simulink model "Auto_mode"  (R2017a)
settings: Solver=VariableStepAuto  StartTime=0.0  StopTime=30  FixedStep=Ts  RelTol=1e-3  EnableMultiTasking=on
model workspace (MAT data in the model file):
  AC_ATTITUDE_ACCEL_Y_CONTROLLER_MAX_RADSS = Simulink.Signal
  AC_ATTITUDE_ACCEL_Y_CONTROLLER_MAX_RADSS.DataType = 'double'
  AC_ATTITUDE_ACCEL_Y_CONTROLLER_MAX_RADSS.Dimensions = 1
  AC_ATTITUDE_ACCEL_Y_CONTROLLER_MAX_RADSS.DimensionsMode = 'auto'
  AC_ATTITUDE_ACCEL_Y_CONTROLLER_MAX_RADSS.Complexity = 'real'
  AC_ATTITUDE_ACCEL_Y_CONTROLLER_MAX_RADSS.SampleTime = -1
  AC_ATTITUDE_ACCEL_Y_CONTROLLER_MAX_RADSS.SamplingMode = 'Sample based'
  AC_ATTITUDE_ACCEL_Y_CONTROLLER_MAX_RADSS.InitialValue = '0.5'
  AC_ATTITUDE_CONTROL_MAX = Simulink.Signal
  AC_ATTITUDE_CONTROL_MAX.DataType = 'double'
  AC_ATTITUDE_CONTROL_MAX.Dimensions = 1
  AC_ATTITUDE_CONTROL_MAX.DimensionsMode = 'auto'
  AC_ATTITUDE_CONTROL_MAX.Complexity = 'real'
  AC_ATTITUDE_CONTROL_MAX.SampleTime = -1
  AC_ATTITUDE_CONTROL_MAX.SamplingMode = 'Sample based'
  AC_ATTITUDE_CONTROL_MAX.InitialValue = '0.5'
  AC_ATTITUDE_THRUST_ERROR_ANGLE = Simulink.Signal
  AC_ATTITUDE_THRUST_ERROR_ANGLE.DataType = 'double'
  AC_ATTITUDE_THRUST_ERROR_ANGLE.Dimensions = 1
  AC_ATTITUDE_THRUST_ERROR_ANGLE.DimensionsMode = 'auto'
  AC_ATTITUDE_THRUST_ERROR_ANGLE.Complexity = 'real'
  AC_ATTITUDE_THRUST_ERROR_ANGLE.SampleTime = -1
  AC_ATTITUDE_THRUST_ERROR_ANGLE.SamplingMode = 'Sample based'
  AC_ATTITUDE_THRUST_ERROR_ANGLE.InitialValue = '1000'
  ROLL_PITCH_INPUT_MAX = Simulink.Signal
  ROLL_PITCH_INPUT_MAX.DataType = 'double'
  ROLL_PITCH_INPUT_MAX.Dimensions = 1
  ROLL_PITCH_INPUT_MAX.DimensionsMode = 'auto'
  ROLL_PITCH_INPUT_MAX.Complexity = 'real'
  ROLL_PITCH_INPUT_MAX.SampleTime = -1
  ROLL_PITCH_INPUT_MAX.SamplingMode = 'Sample based'
  ROLL_PITCH_INPUT_MAX.InitialValue = '3000'
  Sig = Simulink.Signal
  Sig.DataType = 'auto'
  Sig.Dimensions = -1
  Sig.DimensionsMode = 'auto'
  Sig.Complexity = 'auto'
  Sig.SampleTime = -1
  Sig.SamplingMode = 'auto'
  Sig1 = Simulink.Signal
  Sig1.DataType = 'auto'
  Sig1.Dimensions = -1
  Sig1.DimensionsMode = 'auto'
  Sig1.Complexity = 'auto'
  Sig1.SampleTime = -1
  Sig1.SamplingMode = 'auto'
  acro_yaw_p = Simulink.Signal
  acro_yaw_p.DataType = 'double'
  acro_yaw_p.Dimensions = 1
  acro_yaw_p.DimensionsMode = 'auto'
  acro_yaw_p.Complexity = 'real'
  acro_yaw_p.SampleTime = -1
  acro_yaw_p.SamplingMode = 'Sample based'
  acro_yaw_p.InitialValue = '45'
  angle_max = Simulink.Signal
  angle_max.DataType = 'double'
  angle_max.Dimensions = 1
  angle_max.DimensionsMode = 'auto'
  angle_max.Complexity = 'real'
  angle_max.SampleTime = -1
  angle_max.SamplingMode = 'Sample based'
  angle_max.InitialValue = '3000'
  attitude_target_ang_vel = Simulink.Signal
  attitude_target_ang_vel.DataType = 'double'
  attitude_target_ang_vel.Dimensions = 3
  attitude_target_ang_vel.DimensionsMode = 'auto'
  attitude_target_ang_vel.Complexity = 'real'
  attitude_target_ang_vel.SampleTime = -1
  attitude_target_ang_vel.SamplingMode = 'Sample based'
  attitude_target_ang_vel.InitialValue = '[0 0 0]'
  attitude_target_euler_angle_x = Simulink.Signal
  attitude_target_euler_angle_x.DataType = 'double'
  attitude_target_euler_angle_x.Dimensions = 1
  attitude_target_euler_angle_x.DimensionsMode = 'auto'
  attitude_target_euler_angle_x.Complexity = 'real'
  attitude_target_euler_angle_x.SampleTime = -1
  attitude_target_euler_angle_x.SamplingMode = 'Sample based'
  attitude_target_euler_angle_x.InitialValue = '0'
  attitude_target_euler_angle_y = Simulink.Signal
  attitude_target_euler_angle_y.DataType = 'double'
  attitude_target_euler_angle_y.Dimensions = 1
  attitude_target_euler_angle_y.DimensionsMode = 'auto'
  attitude_target_euler_angle_y.Complexity = 'real'
  attitude_target_euler_angle_y.SampleTime = -1
  attitude_target_euler_angle_y.SamplingMode = 'Sample based'
  attitude_target_euler_angle_y.InitialValue = '0'
  attitude_target_euler_angle_z = Simulink.Signal
  attitude_target_euler_angle_z.DataType = 'double'
  attitude_target_euler_angle_z.Dimensions = 1
  attitude_target_euler_angle_z.DimensionsMode = 'auto'
  attitude_target_euler_angle_z.Complexity = 'real'
  attitude_target_euler_angle_z.SampleTime = -1
  attitude_target_euler_angle_z.SamplingMode = 'Sample based'
  attitude_target_euler_angle_z.InitialValue = '0'
  attitude_target_euler_rate = Simulink.Signal
  attitude_target_euler_rate.DataType = 'double'
  attitude_target_euler_rate.Dimensions = 3
  attitude_target_euler_rate.DimensionsMode = 'auto'
  attitude_target_euler_rate.Complexity = 'real'
  attitude_target_euler_rate.SampleTime = -1
  attitude_target_euler_rate.SamplingMode = 'Sample based'
  attitude_target_euler_rate.InitialValue = '[0 0 0]'
  attitude_target_quat = Simulink.Signal
  attitude_target_quat.DataType = 'double'
  attitude_target_quat.Dimensions = 4
  attitude_target_quat.DimensionsMode = 'auto'
  attitude_target_quat.Complexity = 'real'
  attitude_target_quat.SampleTime = -1
  attitude_target_quat.SamplingMode = 'Sample based'
  attitude_target_quat.InitialValue = '[1 0 0 0]'
  attitude_vehicle_quat = Simulink.Signal
  attitude_vehicle_quat.DataType = 'double'
  attitude_vehicle_quat.Dimensions = 4
  attitude_vehicle_quat.DimensionsMode = 'auto'
  attitude_vehicle_quat.Complexity = 'real'
  attitude_vehicle_quat.SampleTime = -1
  attitude_vehicle_quat.SamplingMode = 'Sample based'
  attitude_vehicle_quat.InitialValue = '[1 0 0 0]'
  dt = Simulink.Signal
  dt.DataType = 'double'
  dt.Dimensions = 1
  dt.DimensionsMode = 'auto'
  dt.Complexity = 'real'
  dt.SampleTime = -1
  dt.SamplingMode = 'Sample based'
  dt.InitialValue = '0.01'
  false = 0
  limit_roll_pitch = Simulink.Signal
  limit_roll_pitch.DataType = 'double'
  limit_roll_pitch.Dimensions = 1
  limit_roll_pitch.DimensionsMode = 'auto'
  limit_roll_pitch.Complexity = 'real'
  limit_roll_pitch.SampleTime = -1
  limit_roll_pitch.SamplingMode = 'Sample based'
  limit_roll_pitch.InitialValue = '0.0'
  limit_throttle_upper = Simulink.Signal
  limit_throttle_upper.DataType = 'logical'
  limit_throttle_upper.Dimensions = 1
  limit_throttle_upper.DimensionsMode = 'auto'
  limit_throttle_upper.Complexity = 'real'
  limit_throttle_upper.SampleTime = -1
  limit_throttle_upper.SamplingMode = 'Sample based'
  limit_throttle_upper.InitialValue = '0'
  limit_yaw = Simulink.Signal
  limit_yaw.DataType = 'double'
  limit_yaw.Dimensions = 1
  limit_yaw.DimensionsMode = 'auto'
  limit_yaw.Complexity = 'real'
  limit_yaw.SampleTime = -1
  limit_yaw.SamplingMode = 'Sample based'
  limit_yaw.InitialValue = '0'
  loop_rate = Simulink.Signal
  loop_rate.DataType = 'double'
  loop_rate.Dimensions = 1
  loop_rate.DimensionsMode = 'auto'
  loop_rate.Complexity = 'real'
  loop_rate.SampleTime = -1
  loop_rate.SamplingMode = 'Sample based'
  loop_rate.InitialValue = '100'
  pitch_attitude_kP = Simulink.Signal
  pitch_attitude_kP.DataType = 'double'
  pitch_attitude_kP.Dimensions = 1
  pitch_attitude_kP.DimensionsMode = 'auto'
  pitch_attitude_kP.Complexity = 'real'
  pitch_attitude_kP.SampleTime = -1
  pitch_attitude_kP.SamplingMode = 'Sample based'
  pitch_attitude_kP.InitialValue = '20'
  pitch_factor = Simulink.Signal
  pitch_factor.DataType = 'double'
  pitch_factor.Dimensions = 4
  pitch_factor.DimensionsMode = 'auto'
  pitch_factor.Complexity = 'real'
  pitch_factor.SampleTime = -1
  pitch_factor.SamplingMode = 'Sample based'
  pitch_factor.InitialValue = '[cos(deg2rad(15)) -cos(deg2rad(15)) cos(deg2rad(15)) -cos(deg2rad(15))]'
  pitch_rate_derivative = Simulink.Signal
  pitch_rate_derivative.DataType = 'double'
  pitch_rate_derivative.Dimensions = 1
  pitch_rate_derivative.DimensionsMode = 'auto'
  pitch_rate_derivative.Complexity = 'real'
  pitch_rate_derivative.SampleTime = -1
  pitch_rate_derivative.SamplingMode = 'Sample based'
  pitch_rate_derivative.InitialValue = '0'
  pitch_rate_error_rads = Simulink.Signal
  pitch_rate_error_rads.DataType = 'double'
  pitch_rate_error_rads.Dimensions = 1
  pitch_rate_error_rads.DimensionsMode = 'auto'
  pitch_rate_error_rads.Complexity = 'real'
  pitch_rate_error_rads.SampleTime = -1
  pitch_rate_error_rads.SamplingMode = 'Sample based'
  pitch_rate_error_rads.InitialValue = '0'
  pitch_rate_filt_hz = Simulink.Signal
  pitch_rate_filt_hz.DataType = 'double'
  pitch_rate_filt_hz.Dimensions = 1
  pitch_rate_filt_hz.DimensionsMode = 'auto'
  pitch_rate_filt_hz.Complexity = 'real'
  pitch_rate_filt_hz.SampleTime = -1
  pitch_rate_filt_hz.SamplingMode = 'Sample based'
  pitch_rate_filt_hz.InitialValue = '1/(2*pi)'
  pitch_rate_imax = Simulink.Signal
  pitch_rate_imax.DataType = 'double'
  pitch_rate_imax.Dimensions = 1
  pitch_rate_imax.DimensionsMode = 'auto'
  pitch_rate_imax.Complexity = 'real'
  pitch_rate_imax.SampleTime = -1
  pitch_rate_imax.SamplingMode = 'Sample based'
  pitch_rate_imax.InitialValue = '200'
  pitch_rate_integrator = Simulink.Signal
  pitch_rate_integrator.DataType = 'double'
  pitch_rate_integrator.Dimensions = 1
  pitch_rate_integrator.DimensionsMode = 'auto'
  pitch_rate_integrator.Complexity = 'real'
  pitch_rate_integrator.SampleTime = -1
  pitch_rate_integrator.SamplingMode = 'Sample based'
  pitch_rate_integrator.InitialValue = '0'
  pitch_rate_kD = Simulink.Signal
  pitch_rate_kD.DataType = 'double'
  pitch_rate_kD.Dimensions = 1
  pitch_rate_kD.DimensionsMode = 'auto'
  pitch_rate_kD.Complexity = 'real'
  pitch_rate_kD.SampleTime = -1
  pitch_rate_kD.SamplingMode = 'Sample based'
  pitch_rate_kD.InitialValue = '0.004'
  pitch_rate_kI = Simulink.Signal
  pitch_rate_kI.DataType = 'double'
  pitch_rate_kI.Dimensions = 1
  pitch_rate_kI.DimensionsMode = 'auto'
  pitch_rate_kI.Complexity = 'real'
  pitch_rate_kI.SampleTime = -1
  pitch_rate_kI.SamplingMode = 'Sample based'
  pitch_rate_kI.InitialValue = '0.1'
  pitch_rate_kP = Simulink.Signal
  pitch_rate_kP.DataType = 'double'
  pitch_rate_kP.Dimensions = 1
  pitch_rate_kP.DimensionsMode = 'auto'
  pitch_rate_kP.Complexity = 'real'
  pitch_rate_kP.SampleTime = -1
  pitch_rate_kP.SamplingMode = 'Sample based'
  pitch_rate_kP.InitialValue = '0.5'
  pitch_rate_last_input = Simulink.Signal
  pitch_rate_last_input.DataType = 'double'
  pitch_rate_last_input.Dimensions = 1
  pitch_rate_last_input.DimensionsMode = 'auto'
  pitch_rate_last_input.Complexity = 'real'
  pitch_rate_last_input.SampleTime = -1
  pitch_rate_last_input.SamplingMode = 'Sample based'
  pitch_rate_last_input.InitialValue = '0'
  pitch_rate_proportional = Simulink.Signal
  pitch_rate_proportional.DataType = 'double'
  pitch_rate_proportional.Dimensions = 1
  pitch_rate_proportional.DimensionsMode = 'auto'
  pitch_rate_proportional.Complexity = 'real'
  pitch_rate_proportional.SampleTime = -1
  pitch_rate_proportional.SamplingMode = 'Sample based'
  pitch_rate_proportional.InitialValue = '0'
  pwm_max = Simulink.Signal
  pwm_max.DataType = 'double'
  pwm_max.Dimensions = 1
  pwm_max.DimensionsMode = 'auto'
  pwm_max.Complexity = 'real'
  pwm_max.SampleTime = -1
  pwm_max.SamplingMode = 'Sample based'
  pwm_max.InitialValue = '2000'
  pwm_min = Simulink.Signal
  pwm_min.DataType = 'double'
  pwm_min.Dimensions = 1
  pwm_min.DimensionsMode = 'auto'
  pwm_min.Complexity = 'real'
  pwm_min.SampleTime = -1
  pwm_min.SamplingMode = 'Sample based'
  pwm_min.InitialValue = '1039'
  rate_bf_ff_enabled = Simulink.Signal
  rate_bf_ff_enabled.DataType = 'double'
  rate_bf_ff_enabled.Dimensions = 1
  rate_bf_ff_enabled.DimensionsMode = 'auto'
  rate_bf_ff_enabled.Complexity = 'real'
  rate_bf_ff_enabled.SampleTime = -1
  rate_bf_ff_enabled.SamplingMode = 'Sample based'
  rate_bf_ff_enabled.InitialValue = '0'
  rate_target_ang_vel = Simulink.Signal
  rate_target_ang_vel.DataType = 'double'
  rate_target_ang_vel.Dimensions = 3
  rate_target_ang_vel.DimensionsMode = 'auto'
  rate_target_ang_vel.Complexity = 'real'
  rate_target_ang_vel.SampleTime = -1
  rate_target_ang_vel.SamplingMode = 'Sample based'
  rate_target_ang_vel.InitialValue = '[0 0 0]'
  roll_attitude_kP = Simulink.Signal
  roll_attitude_kP.DataType = 'double'
  roll_attitude_kP.Dimensions = 1
  roll_attitude_kP.DimensionsMode = 'auto'
  roll_attitude_kP.Complexity = 'real'
  roll_attitude_kP.SampleTime = -1
  roll_attitude_kP.SamplingMode = 'Sample based'
  roll_attitude_kP.InitialValue = '20'
  roll_factor = Simulink.Signal
  roll_factor.DataType = 'double'
  roll_factor.Dimensions = 4
  roll_factor.DimensionsMode = 'auto'
  roll_factor.Complexity = 'real'
  roll_factor.SampleTime = -1
  roll_factor.SamplingMode = 'Sample based'
  roll_factor.InitialValue = '[-sin(deg2rad(15)) sin(deg2rad(15)) sin(deg2rad(15)) -sin(deg2rad(15))]'
  roll_rate_derivative = Simulink.Signal
  roll_rate_derivative.DataType = 'double'
  roll_rate_derivative.Dimensions = 1
  roll_rate_derivative.DimensionsMode = 'auto'
  roll_rate_derivative.Complexity = 'real'
  roll_rate_derivative.SampleTime = -1
  roll_rate_derivative.SamplingMode = 'Sample based'
  roll_rate_derivative.InitialValue = '0'
  roll_rate_error_rads = Simulink.Signal
  roll_rate_error_rads.DataType = 'double'
  roll_rate_error_rads.Dimensions = 1
  roll_rate_error_rads.DimensionsMode = 'auto'
  roll_rate_error_rads.Complexity = 'real'
  roll_rate_error_rads.SampleTime = -1
  roll_rate_error_rads.SamplingMode = 'Sample based'
  roll_rate_error_rads.InitialValue = '0'
  roll_rate_filt_hz = Simulink.Signal
  roll_rate_filt_hz.DataType = 'double'
  roll_rate_filt_hz.Dimensions = 1
  roll_rate_filt_hz.DimensionsMode = 'auto'
  roll_rate_filt_hz.Complexity = 'real'
  roll_rate_filt_hz.SampleTime = -1
  roll_rate_filt_hz.SamplingMode = 'Sample based'
  roll_rate_filt_hz.InitialValue = '1/(2*pi)'
  roll_rate_imax = Simulink.Signal
  roll_rate_imax.DataType = 'double'
  roll_rate_imax.Dimensions = 1
  roll_rate_imax.DimensionsMode = 'auto'
  roll_rate_imax.Complexity = 'real'
  roll_rate_imax.SampleTime = -1
  roll_rate_imax.SamplingMode = 'Sample based'
  roll_rate_imax.InitialValue = '200'
  roll_rate_integrator = Simulink.Signal
  roll_rate_integrator.DataType = 'double'
  roll_rate_integrator.Dimensions = 1
  roll_rate_integrator.DimensionsMode = 'auto'
  roll_rate_integrator.Complexity = 'real'
  roll_rate_integrator.SampleTime = -1
  roll_rate_integrator.SamplingMode = 'Sample based'
  roll_rate_integrator.InitialValue = '0'
  roll_rate_kD = Simulink.Signal
  roll_rate_kD.DataType = 'double'
  roll_rate_kD.Dimensions = 1
  roll_rate_kD.DimensionsMode = 'auto'
  roll_rate_kD.Complexity = 'real'
  roll_rate_kD.SampleTime = -1
  roll_rate_kD.SamplingMode = 'Sample based'
  roll_rate_kD.InitialValue = '0.004'
  roll_rate_kI = Simulink.Signal
  roll_rate_kI.DataType = 'double'
  roll_rate_kI.Dimensions = 1
  roll_rate_kI.DimensionsMode = 'auto'
  roll_rate_kI.Complexity = 'real'
  roll_rate_kI.SampleTime = -1
  roll_rate_kI.SamplingMode = 'Sample based'
  roll_rate_kI.InitialValue = '0.1'
  roll_rate_kP = Simulink.Signal
  roll_rate_kP.DataType = 'double'
  roll_rate_kP.Dimensions = 1
  roll_rate_kP.DimensionsMode = 'auto'
  roll_rate_kP.Complexity = 'real'
  roll_rate_kP.SampleTime = -1
  roll_rate_kP.SamplingMode = 'Sample based'
  roll_rate_kP.InitialValue = '1'
  roll_rate_last_input = Simulink.Signal
  roll_rate_last_input.DataType = 'double'
  roll_rate_last_input.Dimensions = 1
  roll_rate_last_input.DimensionsMode = 'auto'
  roll_rate_last_input.Complexity = 'real'
  roll_rate_last_input.SampleTime = -1
  roll_rate_last_input.SamplingMode = 'Sample based'
  roll_rate_last_input.InitialValue = '0'
  roll_rate_proportional = Simulink.Signal
  roll_rate_proportional.DataType = 'double'
  roll_rate_proportional.Dimensions = 1
  roll_rate_proportional.DimensionsMode = 'auto'
  roll_rate_proportional.Complexity = 'real'
  roll_rate_proportional.SampleTime = -1
  roll_rate_proportional.SamplingMode = 'Sample based'
  roll_rate_proportional.InitialValue = '0'
  spin_max = Simulink.Signal
  spin_max.DataType = 'double'
  spin_max.Dimensions = 1
  spin_max.DimensionsMode = 'auto'
  spin_max.Complexity = 'real'
  spin_max.SampleTime = -1
  spin_max.SamplingMode = 'Sample based'
  spin_max.InitialValue = '0.95'
  spin_min = Simulink.Signal
  spin_min.DataType = 'double'
  spin_min.Dimensions = 1
  spin_min.DimensionsMode = 'auto'
  spin_min.Complexity = 'real'
  spin_min.SampleTime = -1
  spin_min.SamplingMode = 'Sample based'
  spin_min.InitialValue = '0.15'
  throttle_avg_max = Simulink.Signal
  throttle_avg_max.DataType = 'double'
  throttle_avg_max.Dimensions = 1
  throttle_avg_max.DimensionsMode = 'auto'
  throttle_avg_max.Complexity = 'real'
  throttle_avg_max.SampleTime = -1
  throttle_avg_max.SamplingMode = 'Sample based'
  throttle_avg_max.InitialValue = '0'
  throttle_filter_cutoff_freq = Simulink.Signal
  throttle_filter_cutoff_freq.DataType = 'double'
  throttle_filter_cutoff_freq.Dimensions = 1
  throttle_filter_cutoff_freq.DimensionsMode = 'auto'
  throttle_filter_cutoff_freq.Complexity = 'real'
  throttle_filter_cutoff_freq.SampleTime = -1
  throttle_filter_cutoff_freq.SamplingMode = 'Sample based'
  throttle_filter_cutoff_freq.InitialValue = '0.5'
  throttle_filter_output = Simulink.Signal
  throttle_filter_output.DataType = 'double'
  throttle_filter_output.Dimensions = 1
  throttle_filter_output.DimensionsMode = 'auto'
  throttle_filter_output.Complexity = 'real'
  throttle_filter_output.SampleTime = -1
  throttle_filter_output.SamplingMode = 'Sample based'
  throttle_filter_output.InitialValue = '0'
  throttle_in = Simulink.Signal
  throttle_in.DataType = 'double'
  throttle_in.Dimensions = 1
  throttle_in.DimensionsMode = 'auto'
  throttle_in.Complexity = 'real'
  throttle_in.SampleTime = -1
  throttle_in.SamplingMode = 'Sample based'
  throttle_in.InitialValue = '0'
  throttle_rpy_mix = Simulink.Signal
  throttle_rpy_mix.DataType = 'double'
  throttle_rpy_mix.Dimensions = 1
  throttle_rpy_mix.DimensionsMode = 'auto'
  throttle_rpy_mix.Complexity = 'real'
  throttle_rpy_mix.SampleTime = -1
  throttle_rpy_mix.SamplingMode = 'Sample based'
  throttle_rpy_mix.InitialValue = '0'
  throttle_rpy_mix_desired = Simulink.Signal
  throttle_rpy_mix_desired.DataType = 'double'
  throttle_rpy_mix_desired.Dimensions = 1
  throttle_rpy_mix_desired.DimensionsMode = 'auto'
  throttle_rpy_mix_desired.Complexity = 'real'
  throttle_rpy_mix_desired.SampleTime = -1
  throttle_rpy_mix_desired.SamplingMode = 'Sample based'
  throttle_rpy_mix_desired.InitialValue = '0'
  throttle_thrust = Simulink.Signal
  throttle_thrust.DataType = 'double'
  throttle_thrust.Dimensions = 1
  throttle_thrust.DimensionsMode = 'auto'
  throttle_thrust.Complexity = 'real'
  throttle_thrust.SampleTime = -1
  throttle_thrust.SamplingMode = 'Sample based'
  throttle_thrust.InitialValue = '0'
  throttle_thrust_best_rpy = Simulink.Signal
  throttle_thrust_best_rpy.DataType = 'double'
  throttle_thrust_best_rpy.Dimensions = 1
  throttle_thrust_best_rpy.DimensionsMode = 'auto'
  throttle_thrust_best_rpy.Complexity = 'real'
  throttle_thrust_best_rpy.SampleTime = -1
  throttle_thrust_best_rpy.SamplingMode = 'Sample based'
  throttle_thrust_best_rpy.InitialValue = '0'
  throttle_thrust_max = Simulink.Signal
  throttle_thrust_max.DataType = 'double'
  throttle_thrust_max.Dimensions = 1
  throttle_thrust_max.DimensionsMode = 'auto'
  throttle_thrust_max.Complexity = 'real'
  throttle_thrust_max.SampleTime = -1
  throttle_thrust_max.SamplingMode = 'Sample based'
  throttle_thrust_max.InitialValue = '1'
  thrust_error_angle = Simulink.Signal
  thrust_error_angle.DataType = 'double'
  thrust_error_angle.Dimensions = 1
  thrust_error_angle.DimensionsMode = 'auto'
  thrust_error_angle.Complexity = 'real'
  thrust_error_angle.SampleTime = -1
  thrust_error_angle.SamplingMode = 'Sample based'
  thrust_error_angle.InitialValue = '0'
  thrust_rpyt_out = Simulink.Signal
  thrust_rpyt_out.DataType = 'double'
  thrust_rpyt_out.Dimensions = 4
  thrust_rpyt_out.DimensionsMode = 'auto'
  thrust_rpyt_out.Complexity = 'real'
  thrust_rpyt_out.SampleTime = -1
  thrust_rpyt_out.SamplingMode = 'Sample based'
  thrust_rpyt_out.InitialValue = '[0 0 0 0]'
  true = 1
  use_ff_and_input_shaping = Simulink.Signal
  use_ff_and_input_shaping.DataType = 'double'
  use_ff_and_input_shaping.Dimensions = 1
  use_ff_and_input_shaping.DimensionsMode = 'auto'
  use_ff_and_input_shaping.Complexity = 'real'
  use_ff_and_input_shaping.SampleTime = -1
  use_ff_and_input_shaping.SamplingMode = 'Sample based'
  use_ff_and_input_shaping.InitialValue = '0'
  variableType = 'S'
  yaw_allowed = Simulink.Signal
  yaw_allowed.DataType = 'double'
  yaw_allowed.Dimensions = 1
  yaw_allowed.DimensionsMode = 'auto'
  yaw_allowed.Complexity = 'real'
  yaw_allowed.SampleTime = -1
  yaw_allowed.SamplingMode = 'Sample based'
  yaw_allowed.InitialValue = '1'
  yaw_attitude_kP = Simulink.Signal
  yaw_attitude_kP.DataType = 'double'
  yaw_attitude_kP.Dimensions = 1
  yaw_attitude_kP.DimensionsMode = 'auto'
  yaw_attitude_kP.Complexity = 'real'
  yaw_attitude_kP.SampleTime = -1
  yaw_attitude_kP.SamplingMode = 'Sample based'
  yaw_attitude_kP.InitialValue = '4.5'
  yaw_factor = Simulink.Signal
  yaw_factor.DataType = 'double'
  yaw_factor.Dimensions = 4
  yaw_factor.DimensionsMode = 'auto'
  yaw_factor.Complexity = 'real'
  yaw_factor.SampleTime = -1
  yaw_factor.SamplingMode = 'Sample based'
  yaw_factor.InitialValue = '[0.1 0.1 -0.1 -0.1]'
  yaw_headroom = Simulink.Signal
  yaw_headroom.DataType = 'double'
  yaw_headroom.Dimensions = 1
  yaw_headroom.DimensionsMode = 'auto'
  yaw_headroom.Complexity = 'real'
  yaw_headroom.SampleTime = -1
  yaw_headroom.SamplingMode = 'Sample based'
  yaw_headroom.InitialValue = '200'
  yaw_rate_derivative = Simulink.Signal
  yaw_rate_derivative.DataType = 'double'
  yaw_rate_derivative.Dimensions = 1
  yaw_rate_derivative.DimensionsMode = 'auto'
  yaw_rate_derivative.Complexity = 'real'
  yaw_rate_derivative.SampleTime = -1
  yaw_rate_derivative.SamplingMode = 'Sample based'
  yaw_rate_derivative.InitialValue = '0'
  yaw_rate_error_rads = Simulink.Signal
  yaw_rate_error_rads.DataType = 'double'
  yaw_rate_error_rads.Dimensions = 1
  yaw_rate_error_rads.DimensionsMode = 'auto'
  yaw_rate_error_rads.Complexity = 'real'
  yaw_rate_error_rads.SampleTime = -1
  yaw_rate_error_rads.SamplingMode = 'Sample based'
  yaw_rate_error_rads.InitialValue = '0'
  yaw_rate_filt_hz = Simulink.Signal
  yaw_rate_filt_hz.DataType = 'double'
  yaw_rate_filt_hz.Dimensions = 1
  yaw_rate_filt_hz.DimensionsMode = 'auto'
  yaw_rate_filt_hz.Complexity = 'real'
  yaw_rate_filt_hz.SampleTime = -1
  yaw_rate_filt_hz.SamplingMode = 'Sample based'
  yaw_rate_filt_hz.InitialValue = '1/(2*pi)'
  yaw_rate_imax = Simulink.Signal
  yaw_rate_imax.DataType = 'double'
  yaw_rate_imax.Dimensions = 1
  yaw_rate_imax.DimensionsMode = 'auto'
  yaw_rate_imax.Complexity = 'real'
  yaw_rate_imax.SampleTime = -1
  yaw_rate_imax.SamplingMode = 'Sample based'
  yaw_rate_imax.InitialValue = '200'
  yaw_rate_integrator = Simulink.Signal
  yaw_rate_integrator.DataType = 'double'
  yaw_rate_integrator.Dimensions = 1
  yaw_rate_integrator.DimensionsMode = 'auto'
  yaw_rate_integrator.Complexity = 'real'
  yaw_rate_integrator.SampleTime = -1
  yaw_rate_integrator.SamplingMode = 'Sample based'
  yaw_rate_integrator.InitialValue = '0'
  yaw_rate_kD = Simulink.Signal
  yaw_rate_kD.DataType = 'double'
  yaw_rate_kD.Dimensions = 1
  yaw_rate_kD.DimensionsMode = 'auto'
  yaw_rate_kD.Complexity = 'real'
  yaw_rate_kD.SampleTime = -1
  yaw_rate_kD.SamplingMode = 'Sample based'
  yaw_rate_kD.InitialValue = '5'
  yaw_rate_kI = Simulink.Signal
  yaw_rate_kI.DataType = 'double'
  yaw_rate_kI.Dimensions = 1
  yaw_rate_kI.DimensionsMode = 'auto'
  yaw_rate_kI.Complexity = 'real'
  yaw_rate_kI.SampleTime = -1
  yaw_rate_kI.SamplingMode = 'Sample based'
  yaw_rate_kI.InitialValue = '0.1'
  yaw_rate_kP = Simulink.Signal
  yaw_rate_kP.DataType = 'double'
  yaw_rate_kP.Dimensions = 1
  yaw_rate_kP.DimensionsMode = 'auto'
  yaw_rate_kP.Complexity = 'real'
  yaw_rate_kP.SampleTime = -1
  yaw_rate_kP.SamplingMode = 'Sample based'
  yaw_rate_kP.InitialValue = '0.2'
  yaw_rate_last_input = Simulink.Signal
  yaw_rate_last_input.DataType = 'double'
  yaw_rate_last_input.Dimensions = 1
  yaw_rate_last_input.DimensionsMode = 'auto'
  yaw_rate_last_input.Complexity = 'real'
  yaw_rate_last_input.SampleTime = -1
  yaw_rate_last_input.SamplingMode = 'Sample based'
  yaw_rate_last_input.InitialValue = '0'
  yaw_rate_proportional = Simulink.Signal
  yaw_rate_proportional.DataType = 'double'
  yaw_rate_proportional.Dimensions = 1
  yaw_rate_proportional.DimensionsMode = 'auto'
  yaw_rate_proportional.Complexity = 'real'
  yaw_rate_proportional.SampleTime = -1
  yaw_rate_proportional.SamplingMode = 'Sample based'
  yaw_rate_proportional.InitialValue = '0'
undefined symbols (not defined in the file or in its folder): Outer_Ts, sensor_max_range, sensor_min_range, Ts
libraries: simulink x8, aerolibactuator x4, vrlib x2, aerolibanim x2, shared6dof x1, aerolibwind2 x1, aerolibnav x1, sharedutil x1, aerolibconvert2 x1, dspbuff3 x1
(part 1 of 2)
settings Model: Creator=s121814  LastModifiedBy=GusBus
settings SolverCC: ZeroCrossControl=DisableAll
settings DataIOCC: SaveFormat=Array  SaveState=on
settings OptimizationCC: LifeSpan=inf
settings DebuggingCC: SFUnexpectedBacktrackingDiag=warning  SFNoUnconditionalDefaultTransitionDiag=warning  SFExecutionAtInitializationDiag=none
settings GRTTargetCC: TargetLangStandard=C89/C90 (ANSI)  GeneratePreprocessorConditionals=Disable all
settings ConfigComp: CovMetricSettings=dw  CovHtmlReporting=on  CovSaveCumulativeToWorkspaceVar=on  CovSaveSingleToWorkspaceVar=on  CovExternalEMLEnable=off

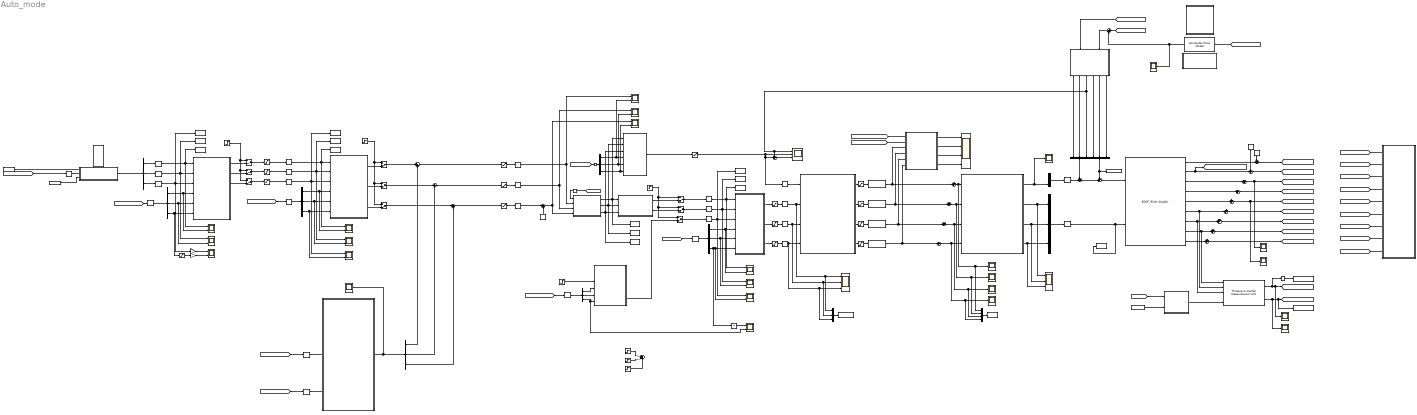
== system Auto_mode ==
  " North" : Scope  NumInputPorts=2
  Altitude : Scope  NumInputPorts=2
  Ameas : Scope
  Body_Accel_X : Scope  NumInputPorts=2
  Body_Accel_Y : Scope  NumInputPorts=2
  Body_Accel_Z : Scope  NumInputPorts=2
  Constant : Constant  Value=-9.81
  Constant1 : Constant  Value=[0 0 9.81]
  Demux{,1..6} (7 alike) : Demux  Outputs=3
  Drag_Concatenate1 : Concatenate  NumInputs=3
  East : Scope  NumInputPorts=2
  Flight Kinematics : shared6dof/6DOF (Euler Angles)  units=Metric (MKS)  mtype=Fixed  rep=Euler Angles  xme_0=[0 0 0]  Vm_0=[0 0 0]  eul_0=[0 0 0]  pm_0=[0 0 0]  mass_0=3.352  mass_e=0.5  mass_f=2.0  inertia=[0.025028 0 0; 0 0.16926 0; 0 0 0.170197]  inertia_e=eye(3)  inertia_f=2*eye(3)  k_quat=1.0  vre_flag=on  abi_flag=on
  Forces : Scope  NumInputPorts=3
  Gain : Gain  Gain=-1
  Gain1 : Gain  Gain=-1
  Global_Vel_X : Scope  NumInputPorts=2
  Global_Vel_Y : Scope  NumInputPorts=2
  Global_Vel_Z : Scope  NumInputPorts=2
  Gravity and Drag Distrubance Calculation : MATLAB Function  TreatAsAtomicUnit=on
  Gravity_Concatenate : Concatenate  NumInputs=3
  Horizontal Wind Model : aerolibwind2/Horizontal Wind Model  units=Metric (MKS)  Vw_source=Internal  Vwind=0  W_source=Internal  Wdeg=297.19390869141
      settings: SourceProductName=Aerospace Blockset  SourceProductBaseCode=AE
  Integrator : Integrator
  Knob : Subsystem  DialogController=hmiCreateDDGDialog  IsWebBlock=on  mask(MWDashboardBlock){webBlockId=fc00fdfc-607d-4439-88d0-141a59e61425, webBlockType=continuousknob, ShowInLibBrowser=on, ShowInitialText=on, HMISrcModelName=Auto_mode}
      mask prompts: webBlockId "WebBlock Id"; webBlockType "WebBlock Type"; HMISrcModelName "Source Model"
      mask help: SimulinkHMI:dialogs:ContinuousKnobDialogDesc
      mask Help: helpview([docroot '/mapfiles/simulink.map'], 'hmi_knob')
      mask Display:
      | if strcmp(get_param(bdroot(gcb),'BlockDiagramType'), 'library')
      |     image([(matlabroot) '/toolbox/simulink/hmi/icons/ContinuousKnob.png']);
      | end
  Linear Second-Order Actuator{1..4} (4 alike) : aerolibactuator/Linear Second-Order Actuator  wn_fin=750  z_fin=1.5  fin_act_0=0  fin_act_vel=0
      settings: SourceProductName=Aerospace Blockset  SourceProductBaseCode=AE
  Linear Velocity Controller : Subsystem
  Manual Switch{,1..5,9..11} (9 alike) : ManualSwitch  CurrentSetting=0
  Measurement Noise6 : simulink/Sources/Band-Limited White Noise  Cov=[0.0025]  Ts=0.25  seed=[23341]
  Measurement Noise7 : simulink/Sources/Band-Limited White Noise  Cov=[0.00000025]  Ts=0.25  seed=[23341]
  Model_Euler : Scope
  Model_Gyro : Scope
  Moments : Scope  NumInputPorts=3
  Motor Mixer : MATLAB Function  TreatAsAtomicUnit=on
  Motor Thrust Calculation : MATLAB Function  TreatAsAtomicUnit=on
  Near Wall Disturbance : MATLAB Function  TreatAsAtomicUnit=on
  Near Wall Effect : Scope  NumInputPorts=4
  Pitch_Rate : Scope  NumInputPorts=2
  Position Controller : Subsystem
  RCOUT{1..4} (4 alike) : Scope
  Rate Controller : Subsystem
  Rocker Switch : Subsystem  DialogController=hmiCreateDDGDialog  IsWebBlock=on  mask(MWDashboardBlock){webBlockId=1389a519-ac27-4032-a6d2-7ec9745cd120, webBlockType=rockerswitch, ShowInLibBrowser=on, ShowInitialText=on, HMISrcModelName=Auto_mode}
      mask prompts: webBlockId "WebBlock Id"; webBlockType "WebBlock Type"; HMISrcModelName "Source Model"
      mask help: SimulinkHMI:dialogs:SwitchDialogDesc
      mask Help: helpview([docroot '/mapfiles/simulink.map'], 'hmi_rocker_switch')
      mask Display:
      | if strcmp(get_param(bdroot(gcb),'BlockDiagramType'), 'library')
      |     image([(matlabroot) '/toolbox/simulink/hmi/icons/RockerSwitch.png']);
      | end
  Roll_Rate : Scope  NumInputPorts=2
  Saturation{,1..4} (5 alike) : Saturate  UpperLimit=5  LowerLimit=-5
  Saturation10 : Saturate  UpperLimit=-10  LowerLimit=-76
  Saturation{11..14} (4 alike) : Saturate  UpperLimit=-6  LowerLimit=-19
  Saturation5 : Saturate  UpperLimit=2  LowerLimit=-2
  Saturation6 : Saturate  UpperLimit=1.5  LowerLimit=-1.5
  Saturation7 : Saturate  UpperLimit=1.5  LowerLimit=-1.5
  Saturation8 : Saturate  UpperLimit=1.5  LowerLimit=-1.5
  Saturation9 : Saturate  UpperLimit=1000  LowerLimit=-5000
  Sensor Implementation : Subsystem
  Slider : Subsystem  DialogController=hmiCreateDDGDialog  IsWebBlock=on  mask(MWDashboardBlock){webBlockId=0b082275-57e0-496a-b4e5-313843d60723, webBlockType=slider, ShowInLibBrowser=on, ShowInitialText=on, HMISrcModelName=Auto_mode}
      mask prompts: webBlockId "WebBlock Id"; webBlockType "WebBlock Type"; HMISrcModelName "Source Model"
      mask help: SimulinkHMI:dialogs:SliderDialogDesc
      mask Help: helpview([docroot '/mapfiles/simulink.map'], 'hmi_slider')
      mask Display:
      | if strcmp(get_param(bdroot(gcb),'BlockDiagramType'), 'library')
      |     image([(matlabroot) '/toolbox/simulink/hmi/icons/Slider.png']);
      | end
  Step1 : Step  Time=4  After=deg2rad(180)  SampleTime=0
  Step3 : Step  After=-1  SampleTime=0
  Step4 : Step  Time=4  After=-0.1  SampleTime=0
  Step5 : Step  After=0.18  SampleTime=0
  Step6 : Step  After=-1  SampleTime=0
  Step7 : Step  Time=8  After=0.2  SampleTime=0
  Step8 : Step  Time=16  After=-0.1  SampleTime=0
  Sum{,14,19..21} (5 alike) : Sum  Inputs=|++
  Sum{1..11,13} (12 alike) : Sum  Inputs=++|
  Sum12 : Sum  Inputs=|+++
  Sum{15..18} (4 alike) : Sum  Inputs=-+|
  Three-axis Inertial Measurement Unit : aerolibnav/Three-axis Inertial Measurement Unit  units=Metric (MKS)  imu=[0 0 0]  i_Ts=0  dtype_a=on  w_a=190  z_a=0.707  a_sf_cc=[1 0 0; 0 1 0; 0 0 1]  a_bias=[0 0 0]  a_sat="[-inf  -inf  -inf  inf inf inf]"  dtype_g=on  w_g=190  z_g=0.707  g_sf_cc=[1 0 0; 0 1 0; 0 0 1]  g_bias=[0 0 0]  g_sens=[0 0 0]  g_sat="[-inf  -inf  -inf  inf inf inf]"  i_rand=on  i_seeds=[23093 23094 23095 23096 23097 23098]  i_pow=[0.001 0.001 0.001 0.0001 0.0001 0.0001]
  Thrust Controller : Subsystem
  Tilt Angle Controller : Subsystem
  To Workspace : ToWorkspace  VariableName=drag_body_force  SaveFormat=Timeseries  SampleTime=-1
  To Workspace and Graphics : Subsystem
  To Workspace1 : ToWorkspace  VariableName=refrollrate  SampleTime=-1
  To Workspace10 : ToWorkspace  VariableName=motor_thrust  SaveFormat=Timeseries  SampleTime=-1
  To Workspace11 : ToWorkspace  VariableName=moments  SampleTime=-1
  To Workspace12 : ToWorkspace  VariableName=refxvel_e  SampleTime=-1
  To Workspace13 : ToWorkspace  VariableName=refyvel_e  SampleTime=-1
  To Workspace14 : ToWorkspace  VariableName=refzvel_e  SampleTime=-1
  To Workspace15 : ToWorkspace  VariableName=torque_requests  SaveFormat=Timeseries  SampleTime=-1
  To Workspace16 : ToWorkspace  VariableName=accelerometer_readings  SaveFormat=Timeseries  SampleTime=-1
  To Workspace17 : ToWorkspace  VariableName=gyroscope_readings  SaveFormat=Timeseries  SampleTime=-1
  To Workspace2 : ToWorkspace  VariableName=refpitchrate  SampleTime=-1
  To Workspace3 : ToWorkspace  VariableName=refxaccel  SampleTime=-1
  To Workspace4 : ToWorkspace  VariableName=refyaccel  SampleTime=-1
  To Workspace5 : ToWorkspace  VariableName=refzaccel  SampleTime=-1
  To Workspace6 : ToWorkspace  VariableName=refyawrate  SampleTime=-1
  To Workspace7 : ToWorkspace  VariableName=refxpos  SampleTime=-1
  To Workspace8 : ToWorkspace  VariableName=refypos  SampleTime=-1
  To Workspace9 : ToWorkspace  VariableName=refzpos  SampleTime=-1
  Torque_Requests : Scope  NumInputPorts=3
  VWind : Scope
  Vector Concatenate : Concatenate  NumInputs=4
  Vector Concatenate2 : Concatenate  NumInputs=3
  Vector Concatenate1 : Concatenate  NumInputs=3
  Vector Concatenate7 : Concatenate  NumInputs=3
  Vector Rotation Body to Earth Acceleration2 : Subsystem
  Vector Rotation Earth to Body Acceleration Desired : Subsystem
  Waypoint Generator NED : Subsystem
  Wmeas : Scope
  Yaw Controller : Subsystem
  Yaw_Angle : Scope  NumInputPorts=2
  Yaw_Rate : Scope  NumInputPorts=2
  ZOH : ZeroOrderHold  SampleTime=Ts
  ZOH1 : ZeroOrderHold  SampleTime=Ts
  ZOH2 : ZeroOrderHold  SampleTime=Ts
  Z_Force : Scope
  Zero-Order Hold{1,5..6,8..10,15..22} (14 alike) : ZeroOrderHold  SampleTime=Ts
  Zero-Order Hold{2..4,7,11..14,23..25} (11 alike) : ZeroOrderHold  SampleTime=Outer_Ts
  pop next way point : Constant  Value=0
  proximity_vector : Scope
  way_point1 : FromWorkspace  VariableName=waypoint_ned  SampleTime=0  Interpolate=off  OutputAfterFinalValue=Holding final value
  tag scope: acceleromter_readings=global, body_linear_acceleration=global, body_linear_velocity=global, body_rotational_acceleration=global, body_rotational_velocity=global, dcm_body_earth=global, earth_linear_acceleration=global, earth_linear_position=global, earth_linear_position_absolute=global, earth_linear_velocity=global, euler_angles_rad=global, gyroscope_readings=global
  wires:
  [body_rotational_velocity] -> To Workspace and Graphics/5(body_rotational_velocity)
  [body_linear_acceleration] -> To Workspace and Graphics/7(body_linear_acceleration)
  [body_rotational_acceleration] -> To Workspace and Graphics/6(body_rotational_acceleration)
  [body_linear_velocity] -> To Workspace and Graphics/4(body_linear_velocity)
  [dcm_body_earth] -> To Workspace and Graphics/3(dcm_body_earth)
  [euler_angles_rad] -> To Workspace and Graphics/2(euler_angles_rad)
  [earth_linear_position] -> To Workspace and Graphics/1(earth_linear_position)
  Sum7/1 -> [earth_linear_velocity]  "earth_linear_velocity"
  Sum6/1 -> [body_rotational_acceleration]  "body_rotational_acceleration"
  Sum8/1 -> [body_linear_acceleration]  "body_linear_acceleration"
  Vector Concatenate7/1 -> Zero-Order Hold5/1
  Sum10/1 -> Model_Euler/1, [euler_angles_rad]  "euler_angles_rad"
  Flight Kinematics/3 -> Sum10/2
  Sum9/1 -> [earth_linear_position]  "earth_linear_position"
  Flight Kinematics/2 -> [earth_linear_position_absolute], Sum9/2
  Flight Kinematics/6 -> Three-axis Inertial Measurement Unit/2, Sum5/2
  Sum5/1 -> [body_rotational_velocity]  "body_rotational_velocity"
  Flight Kinematics/1 -> Sum7/2
  Rate Controller/1(Torque Phi) -> Saturation/1  "roll"
  Rate Controller/2(Torque Theta) -> Saturation1/1  "pitch"
  Rate Controller/3(Torque Psi) -> Saturation5/1  "yaw"
  Demux/1 -> Roll_Rate/2, Rate Controller/4(roll_rate_current)  "actual"
  [gyroscope_readings] -> Zero-Order Hold1/1
  Zero-Order Hold1/1 -> Demux/1
  Vector Concatenate1/1 -> Zero-Order Hold6/1
  Zero-Order Hold5/1 -> Flight Kinematics/2, To Workspace11/1
  Sum13/1 -> Flight Kinematics/1  "Forces"
  Zero-Order Hold2/1 -> Position Controller/1(x_pos_target), To Workspace7/1, " North"/1  "desired"
  Zero-Order Hold3/1 -> Position Controller/2(y_pos_target), To Workspace8/1, East/1  "desired"
  Zero-Order Hold4/1 -> Position Controller/3(z_pos_target), To Workspace9/1, Gain/1
  [earth_linear_position] -> Zero-Order Hold14/1
  Demux2/2 -> East/2, Position Controller/5(y_pos_current)  "actual"
  Demux2/1 -> " North"/2, Position Controller/4(x_pos_current)  "actual"
  Demux2/3 -> Saturation9/1, Position Controller/6(z_pos_current)
  Manual Switch4/1 -> Zero-Order Hold8/1
  Manual Switch3/1 -> Zero-Order Hold9/1
  Saturation2/1 -> Zero-Order Hold19/1
  Saturation3/1 -> Zero-Order Hold18/1
  Saturation4/1 -> Zero-Order Hold17/1
  Manual Switch5/1 -> Zero-Order Hold10/1
  Zero-Order Hold14/1 -> Demux2/1
  Step3/1 -> Manual Switch1/1, Manual Switch/1, Manual Switch2/1
  Demux6/2 -> Sum20/2
  Demux6/1 -> Sum19/2
  Demux6/3 -> Sum21/2
  Linear Velocity Controller/1(x_accel_desired_earth) -> Manual Switch1/2
  Linear Velocity Controller/2(y_accel_desired_earth) -> Manual Switch/2
  Linear Velocity Controller/3(z_accel_desired_earth) -> Manual Switch2/2
  Tilt Angle Controller/2(desired_pitch_rate_rad/s) -> Manual Switch3/2
  Step5/1 -> Manual Switch4/1, Manual Switch3/1, Manual Switch5/1
  Tilt Angle Controller/1(deired_roll_rate_rad/s) -> Manual Switch4/2
  Thrust Controller/1(Z) -> Saturation10/1  "controller"
  [earth_linear_velocity] -> Zero-Order Hold7/1
  Demux3/2 -> Linear Velocity Controller/5(y_vel_current_earth), Global_Vel_Y/2  "actual"
  Demux3/1 -> Linear Velocity Controller/4(x_vel_current_earth), Global_Vel_X/2  "actual"
  Demux3/3 -> Linear Velocity Controller/6(z_vel_current_earth), Global_Vel_Z/2  "climb_rate"
  Zero-Order Hold7/1 -> Demux3/1
  Manual Switch9/1 -> Saturation7/1
  Manual Switch11/1 -> Saturation8/1
  Manual Switch10/1 -> Saturation6/1
  Zero-Order Hold11/1 -> Linear Velocity Controller/1(x_vel_target_earth), To Workspace12/1, Global_Vel_X/1  "desired"
  Zero-Order Hold13/1 -> Linear Velocity Controller/3(z_vel_target_earth), To Workspace14/1, Global_Vel_Z/1  "desired"
  Step6/1 -> Manual Switch9/1, Manual Switch11/1, Manual Switch10/1
  Zero-Order Hold6/1 -> Sum1/2  "Forces"
  Gravity and Drag Distrubance Calculation/6(FDz) -> Drag_Concatenate1/3  "force_drag_z"
  Gravity and Drag Distrubance Calculation/2(FGy) -> Gravity_Concatenate/2  "force_gravity_y"
  Sum3/1 -> [dcm_body_earth]  "dcm_body_earth"
  Gravity and Drag Distrubance Calculation/1(FGx) -> Gravity_Concatenate/1  "force_gravity_x"
  Sum4/1 -> Model_Gyro/1, [body_linear_velocity]  "body_linear_velocity"
  Gravity and Drag Distrubance Calculation/3(FGz) -> Forces/1, Sum2/1, Gravity_Concatenate/3  "force_gravity_z"
  Gravity and Drag Distrubance Calculation/4(FDx) -> Drag_Concatenate1/1  "force_drag_x"
  Gravity and Drag Distrubance Calculation/5(FDy) -> Drag_Concatenate1/2  "force_drag_y"
  Gravity_Concatenate/1 -> Sum1/1
  Position Controller/1(x_vel_desired_earth) -> Manual Switch10/2
  Position Controller/2(y_vel_desired_earth) -> Manual Switch9/2
  Zero-Order Hold8/1 -> To Workspace1/1, Roll_Rate/1, Rate Controller/1(roll_rate_target)  "desired"
  Zero-Order Hold12/1 -> Linear Velocity Controller/2(y_vel_target_earth), To Workspace13/1, Global_Vel_Y/1  "desired"
  Sum2/1 -> Forces/3  "total"
  Zero-Order Hold19/1 -> Vector Rotation Earth to Body Acceleration Desired/2(vectorx_frame1), Body_Accel_X/1  "desired"
  Zero-Order Hold18/1 -> Vector Rotation Earth to Body Acceleration Desired/3(vectory_frame1), Body_Accel_Y/1  "desired"
  Sum/1 -> Vector Rotation Earth to Body Acceleration Desired/4(vectorz_frame1), Body_Accel_Z/1  "desired"
  [dcm_body_earth] -> ZOH/1
  Zero-Order Hold17/1 -> Sum/1
  Constant/1 -> Sum/2
  Flight Kinematics/4 -> Sum3/2
  Flight Kinematics/5 -> Sum4/2
  Flight Kinematics/7 -> Three-axis Inertial Measurement Unit/3, Sum6/2
  Flight Kinematics/8 -> Three-axis Inertial Measurement Unit/1, Sum8/2
  Position Controller/3(z_vel_desired_earth) -> Manual Switch11/2
  Demux4/2 -> Thrust Controller/5(current_accel_y_body), Body_Accel_Y/2  "actual"
  Demux4/1 -> Thrust Controller/4(current_accel_x_body), Body_Accel_X/2  "actual"
  ZOH1/1 -> Demux4/1
  Demux4/3 -> Thrust Controller/6(current_accel_z_body), Body_Accel_Z/2  "actual"
  Vector Rotation Earth to Body Acceleration Desired/1(vectorx_frame2) -> Thrust Controller/1(desired_accel_x_body), To Workspace3/1, Tilt Angle Controller/1(desired_accel_x_body)
  Vector Rotation Earth to Body Acceleration Desired/2(vectory_frame2) -> Thrust Controller/2(desired_accel_y_body), To Workspace4/1, Tilt Angle Controller/2(desired_accel_y_body)
  Vector Rotation Earth to Body Acceleration Desired/3(vectorz_frame2) -> Thrust Controller/3(desired_accel_z_body), To Workspace5/1, Tilt Angle Controller/3(desired_accel_z_body)
  Sum11/1 -> [earth_linear_acceleration]  "earth_linear_acceleration"
  Step8/1 -> Sum12/3
  Step7/1 -> Sum12/2
  Step4/1 -> Sum12/1
  ZOH/1 -> Vector Rotation Earth to Body Acceleration Desired/1(dcm_12)
  Zero-Order Hold10/1 -> To Workspace6/1, Yaw_Rate/1, Rate Controller/3(yaw_rate_target)  "desired"
  Demux/2 -> Rate Controller/5(pitch_rate_current), Pitch_Rate/2  "actual"
  Zero-Order Hold9/1 -> To Workspace2/1, Rate Controller/2(pitch_rate_target), Pitch_Rate/1  "desired"
  Demux/3 -> Integrator/1, Rate Controller/6(yaw_rate_current), Yaw_Rate/2  "actual"
  Sum1/1 -> Sum13/2  "Forces"
  Saturation6/1 -> Zero-Order Hold11/1
  Saturation7/1 -> Zero-Order Hold12/1
  Saturation8/1 -> Zero-Order Hold13/1
  [earth_linear_acceleration] -> To Workspace and Graphics/8(earth_linear_acceleration)
  [earth_linear_velocity] -> To Workspace and Graphics/9(earth_linear_velocity)
  Measurement Noise7/1 -> Sum7/1
  [dcm_body_earth] -> Gravity and Drag Distrubance Calculation/1(DCMeb)
  [body_linear_velocity] -> Sum14/1
  Flight Kinematics/9 -> Sum11/2
  Measurement Noise6/1 -> Sum9/1
  Three-axis Inertial Measurement Unit/2 -> To Workspace17/1, [gyroscope_readings], Wmeas/1
  Three-axis Inertial Measurement Unit/1 -> ZOH2/1, [acceleromter_readings], Ameas/1
  [acceleromter_readings] -> ZOH1/1
  Saturation10/1 -> Forces/2, Zero-Order Hold15/1, Sum2/2
  [dcm_body_earth] -> Vector Rotation Body to Earth Acceleration2/1(dcm_12)
  Constant1/1 -> Vector Rotation Body to Earth Acceleration2/2(vector_frame1)
  Vector Rotation Body to Earth Acceleration2/1(vector_frame2) -> Three-axis Inertial Measurement Unit/5
  Saturation9/1 -> Gain1/1
  Drag_Concatenate1/1 -> Sum13/1, To Workspace/1
  [dcm_body_earth] -> Horizontal Wind Model/1
  Horizontal Wind Model/1 -> VWind/1, Sum14/2
  Sum14/1 -> Gravity and Drag Distrubance Calculation/2(Vb)
  Gain/1 -> Altitude/1  "desired"
  Gain1/1 -> Altitude/2  "actual"
  Motor Thrust Calculation/1(Z) -> Z_Force/1, Vector Concatenate1/3
  Motor Thrust Calculation/2(L) -> Moments/1, Vector Concatenate7/1  "L"
  Motor Thrust Calculation/3(M) -> Moments/2, Vector Concatenate7/2  "M"
  Motor Thrust Calculation/4(N) -> Moments/3, Vector Concatenate7/3  "N"
  Saturation11/1 -> Linear Second-Order Actuator1/1
  Motor Mixer/4(T4) -> Saturation11/1  "rcout4"
  Saturation12/1 -> Linear Second-Order Actuator2/1  "rcout3"
  Saturation13/1 -> Linear Second-Order Actuator3/1  "rcout2"
  Saturation14/1 -> Linear Second-Order Actuator4/1  "rcout1"
  Motor Mixer/3(T3) -> Saturation12/1  "rcout3"
  Motor Mixer/2(T2) -> Saturation13/1  "rcout2"
  Motor Mixer/1(T1) -> Saturation14/1  "rcout1"
  Sum18/1 -> Vector Concatenate/4, RCOUT4/1, Motor Thrust Calculation/4(T4)
  Sum17/1 -> Vector Concatenate/3, RCOUT3/1, Motor Thrust Calculation/3(T3)
  Sum16/1 -> Vector Concatenate/2, RCOUT2/1, Motor Thrust Calculation/2(T2)
  Sum15/1 -> Vector Concatenate/1, RCOUT1/1, Motor Thrust Calculation/1(T1)
  Zero-Order Hold15/1 -> Motor Mixer/1(Z)
  Zero-Order Hold16/1 -> Motor Mixer/2(phi), Vector Concatenate2/1, Torque_Requests/1  "phi"
  Zero-Order Hold20/1 -> Motor Mixer/3(theta), Vector Concatenate2/2, Torque_Requests/2  "theta"
  Zero-Order Hold21/1 -> Vector Concatenate2/3, Torque_Requests/3, Motor Mixer/4(psi)  "psi"
  Saturation/1 -> Zero-Order Hold16/1
  Saturation1/1 -> Zero-Order Hold20/1
  Saturation5/1 -> Zero-Order Hold21/1
  Vector Concatenate/1 -> To Workspace10/1
  Vector Concatenate2/1 -> To Workspace15/1
  ZOH2/1 -> To Workspace16/1
  Step1/1 -> Yaw Controller/3(yaw_angle_target)
  Yaw Controller/3(Psi Rate Target) -> Manual Switch5/2
  Demux1/3 -> Yaw_Angle/2, Yaw Controller/6(yaw_angle_current)
  [euler_angles_rad] -> Zero-Order Hold22/1
  Demux1/2 -> Yaw Controller/5(pitch_rate_current)
  Demux1/1 -> Yaw Controller/4(roll_rate_current)
  Integrator/1 -> Yaw_Angle/1
  Zero-Order Hold22/1 -> Demux1/1
  way_point1/1 -> Waypoint Generator NED/1(list_of_waypoints)
  [earth_linear_position] -> Zero-Order Hold23/1
  Zero-Order Hold23/1 -> Waypoint Generator NED/2(current_pos)
  Waypoint Generator NED/1(current_waypoint) -> Demux5/1
  Demux5/3 -> Zero-Order Hold4/1
  Demux5/1 -> Zero-Order Hold2/1
  Demux5/2 -> Zero-Order Hold3/1
  Linear Second-Order Actuator4/1 -> Near Wall Disturbance/3(T1), Sum15/2
  Linear Second-Order Actuator3/1 -> Near Wall Disturbance/4(T2), Sum16/2
  Linear Second-Order Actuator2/1 -> Near Wall Disturbance/5(T3), Sum17/2
  Linear Second-Order Actuator1/1 -> Near Wall Disturbance/6(T4), Sum18/2
  Near Wall Disturbance/4(Tnw4) -> Near Wall Effect/4
  Near Wall Disturbance/3(Tnw3) -> Near Wall Effect/3
  Near Wall Disturbance/2(Tnw2) -> Near Wall Effect/2
  Near Wall Disturbance/1(Tnw1) -> Near Wall Effect/1
  Sensor Implementation/1(proximity_vector) -> Demux6/1, proximity_vector/1
  [earth_linear_position] -> Zero-Order Hold24/1
  [dcm_body_earth] -> Zero-Order Hold25/1
  Zero-Order Hold24/1 -> Sensor Implementation/2(global position)
  Zero-Order Hold25/1 -> Sensor Implementation/3(dcm)
  Sum20/1 -> Saturation3/1
  Manual Switch/1 -> Sum20/1
  Manual Switch1/1 -> Sum19/1
  Sum19/1 -> Saturation2/1
  Manual Switch2/1 -> Sum21/1
  Sum21/1 -> Saturation4/1
  pop next way point/1 -> Waypoint Generator NED/3(pop)
  [earth_linear_position_absolute] -> Near Wall Disturbance/1(earth_linear_position_absolute)
  [dcm_body_earth] -> Near Wall Disturbance/2(dcm)

== system Auto_mode/Knob ==

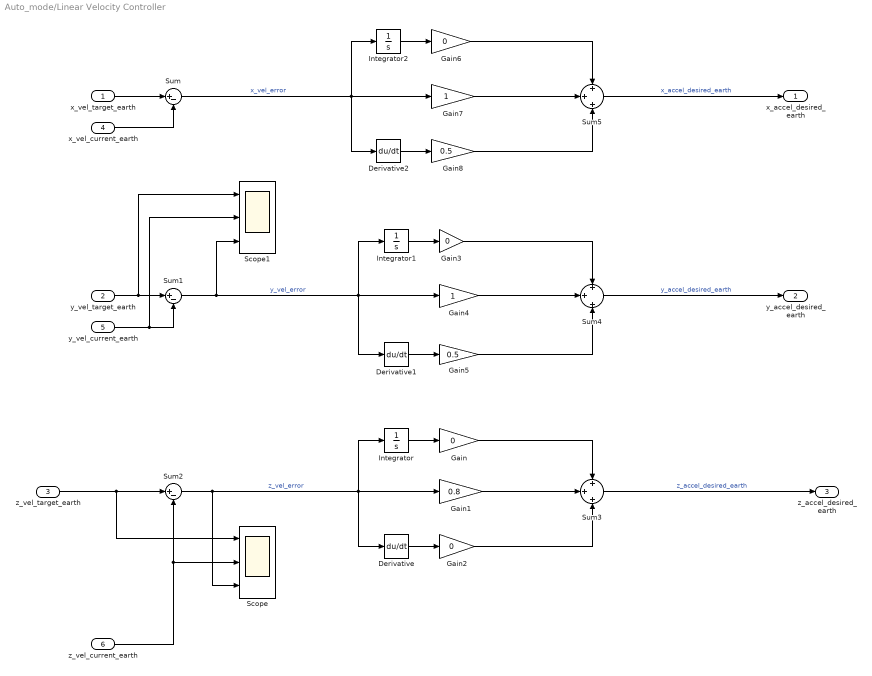
== system Auto_mode/Linear Velocity Controller ==
  x_vel_target_earth : Inport
  y_vel_target_earth : Inport  Port=2
  z_vel_target_earth : Inport  Port=3
  x_vel_current_earth : Inport  Port=4
  y_vel_current_earth : Inport  Port=5
  z_vel_current_earth : Inport  Port=6
  Derivative : Derivative
  Derivative1 : Derivative
  Derivative2 : Derivative
  Gain{,2..3,6} (4 alike) : Gain  Gain=0
  Gain1 : Gain  Gain=0.8
  Gain4 : Gain
  Gain5 : Gain  Gain=0.5
  Gain7 : Gain
  Gain8 : Gain  Gain=0.5
  Integrator : Integrator
  Integrator1 : Integrator
  Integrator2 : Integrator
  Scope : Scope  NumInputPorts=3
  Scope1 : Scope  NumInputPorts=3
  Sum : Sum  Inputs=|+-
  Sum1 : Sum  Inputs=|+-
  Sum2 : Sum  Inputs=|+-
  Sum3 : Sum  Inputs=+|+|+
  Sum4 : Sum  Inputs=+|+|+
  Sum5 : Sum  Inputs=+|+|+
  x_accel_desired_earth : Outport
  y_accel_desired_earth : Outport  Port=2
  z_accel_desired_earth : Outport  Port=3
  wires:
  x_vel_target_earth/1 -> Sum/1
  x_vel_current_earth/1 -> Sum/2
  y_vel_current_earth/1 -> Scope1/2, Sum1/2
  z_vel_target_earth/1 -> Scope/1, Sum2/1
  z_vel_current_earth/1 -> Scope/2, Sum2/2
  Sum3/1 -> z_accel_desired_earth/1  "z_accel_desired_earth"
  Derivative/1 -> Gain2/1
  Gain2/1 -> Sum3/3
  Gain/1 -> Sum3/1
  Integrator/1 -> Gain/1
  Sum2/1 -> Scope/3, Integrator/1, Derivative/1, Gain1/1  "z_vel_error"
  Derivative1/1 -> Gain5/1
  Gain5/1 -> Sum4/3
  Gain4/1 -> Sum4/2
  Gain3/1 -> Sum4/1
  Integrator1/1 -> Gain3/1
  Sum1/1 -> Scope1/3, Integrator1/1, Derivative1/1, Gain4/1  "y_vel_error"
  Sum4/1 -> y_accel_desired_earth/1  "y_accel_desired_earth"
  Derivative2/1 -> Gain8/1
  Gain8/1 -> Sum5/3
  Gain7/1 -> Sum5/2
  Gain6/1 -> Sum5/1
  Integrator2/1 -> Gain6/1
  Sum/1 -> Integrator2/1, Derivative2/1, Gain7/1  "x_vel_error"
  Sum5/1 -> x_accel_desired_earth/1  "x_accel_desired_earth"
  Gain1/1 -> Sum3/2
  y_vel_target_earth/1 -> Scope1/1, Sum1/1

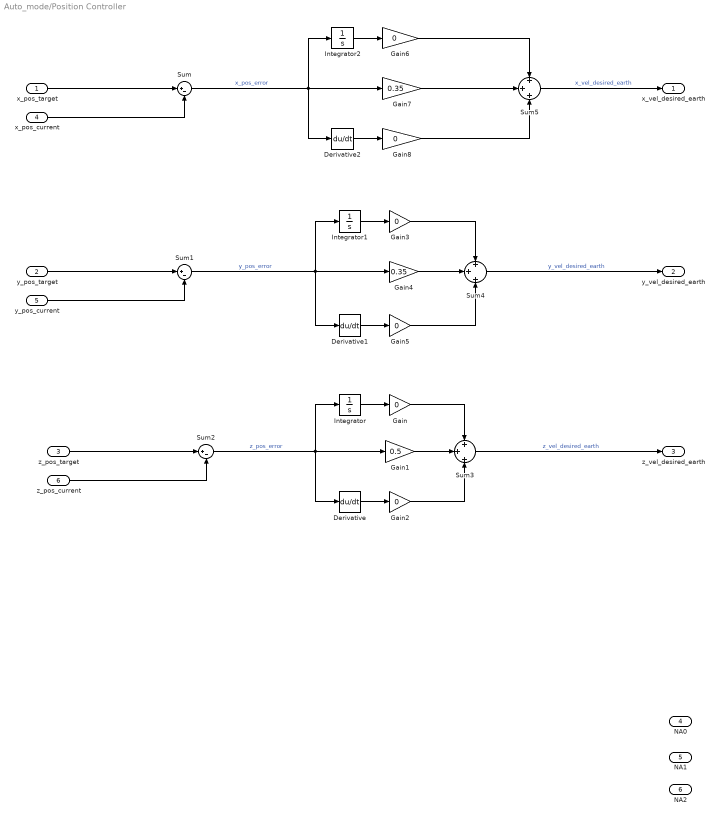
== system Auto_mode/Position Controller ==
  x_pos_target : Inport
  y_pos_target : Inport  Port=2
  z_pos_target : Inport  Port=3
  x_pos_current : Inport  Port=4
  y_pos_current : Inport  Port=5
  z_pos_current : Inport  Port=6
  Derivative : Derivative
  Derivative1 : Derivative
  Derivative2 : Derivative
  Gain{,2..3,5..6,8} (6 alike) : Gain  Gain=0
  Gain1 : Gain  Gain=0.5
  Gain4 : Gain  Gain=0.35
  Gain7 : Gain  Gain=0.35
  Integrator : Integrator
  Integrator1 : Integrator
  Integrator2 : Integrator
  Sum : Sum  Inputs=|+-
  Sum1 : Sum  Inputs=|+-
  Sum2 : Sum  Inputs=|+-
  Sum3 : Sum  Inputs=+|+|+
  Sum4 : Sum  Inputs=+|+|+
  Sum5 : Sum  Inputs=+|+|+
  x_vel_desired_earth : Outport
  y_vel_desired_earth : Outport  Port=2
  z_vel_desired_earth : Outport  Port=3
  NA0 : Outport  Port=4
  NA1 : Outport  Port=5
  NA2 : Outport  Port=6
  wires:
  x_pos_target/1 -> Sum/1
  x_pos_current/1 -> Sum/2
  y_pos_target/1 -> Sum1/1
  y_pos_current/1 -> Sum1/2
  z_pos_target/1 -> Sum2/1
  z_pos_current/1 -> Sum2/2
  Sum3/1 -> z_vel_desired_earth/1  "z_vel_desired_earth"
  Derivative/1 -> Gain2/1
  Gain2/1 -> Sum3/3
  Gain1/1 -> Sum3/2
  Gain/1 -> Sum3/1
  Integrator/1 -> Gain/1
  Sum2/1 -> Integrator/1, Derivative/1, Gain1/1  "z_pos_error"
  Derivative1/1 -> Gain5/1
  Gain5/1 -> Sum4/3
  Gain4/1 -> Sum4/2
  Gain3/1 -> Sum4/1
  Integrator1/1 -> Gain3/1
  Sum1/1 -> Integrator1/1, Derivative1/1, Gain4/1  "y_pos_error"
  Sum4/1 -> y_vel_desired_earth/1  "y_vel_desired_earth"
  Derivative2/1 -> Gain8/1
  Gain8/1 -> Sum5/3
  Gain7/1 -> Sum5/2
  Gain6/1 -> Sum5/1
  Integrator2/1 -> Gain6/1
  Sum/1 -> Integrator2/1, Derivative2/1, Gain7/1  "x_pos_error"
  Sum5/1 -> x_vel_desired_earth/1  "x_vel_desired_earth"

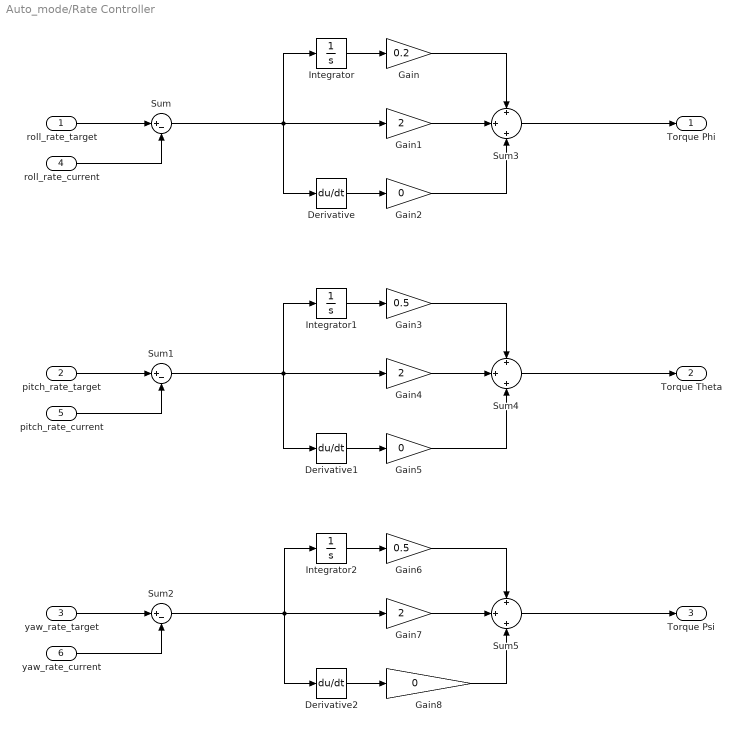
== system Auto_mode/Rate Controller ==
  roll_rate_target : Inport
  pitch_rate_target : Inport  Port=2
  yaw_rate_target : Inport  Port=3
  roll_rate_current : Inport  Port=4
  pitch_rate_current : Inport  Port=5
  yaw_rate_current : Inport  Port=6
  Derivative : Derivative
  Derivative1 : Derivative
  Derivative2 : Derivative
  Gain : Gain  Gain=0.2
  Gain1 : Gain  Gain=2
  Gain2 : Gain  Gain=0
  Gain3 : Gain  Gain=0.5
  Gain4 : Gain  Gain=2
  Gain5 : Gain  Gain=0
  Gain6 : Gain  Gain=0.5
  Gain7 : Gain  Gain=2
  Gain8 : Gain  Gain=0
  Integrator : Integrator
  Integrator1 : Integrator
  Integrator2 : Integrator
  Sum : Sum  Inputs=|+-
  Sum1 : Sum  Inputs=|+-
  Sum2 : Sum  Inputs=|+-
  Sum3 : Sum  Inputs=+|+|+
  Sum4 : Sum  Inputs=+|+|+
  Sum5 : Sum  Inputs=+|+|+
  Torque Phi : Outport
  Torque Theta : Outport  Port=2
  Torque Psi : Outport  Port=3
  wires:
  roll_rate_target/1 -> Sum/1
  roll_rate_current/1 -> Sum/2
  pitch_rate_target/1 -> Sum1/1
  pitch_rate_current/1 -> Sum1/2
  yaw_rate_target/1 -> Sum2/1
  yaw_rate_current/1 -> Sum2/2
  Sum4/1 -> Torque Theta/1
  Sum3/1 -> Torque Phi/1
  Derivative/1 -> Gain2/1
  Gain2/1 -> Sum3/3
  Gain1/1 -> Sum3/2
  Gain/1 -> Sum3/1
  Integrator/1 -> Gain/1
  Sum/1 -> Derivative/1, Integrator/1, Gain1/1
  Derivative1/1 -> Gain5/1
  Gain5/1 -> Sum4/3
  Gain4/1 -> Sum4/2
  Gain3/1 -> Sum4/1
  Integrator1/1 -> Gain3/1
  Sum1/1 -> Derivative1/1, Integrator1/1, Gain4/1
  Sum5/1 -> Torque Psi/1
  Derivative2/1 -> Gain8/1
  Gain8/1 -> Sum5/3
  Gain7/1 -> Sum5/2
  Gain6/1 -> Sum5/1
  Integrator2/1 -> Gain6/1
  Sum2/1 -> Gain7/1, Derivative2/1, Integrator2/1

== system Auto_mode/Rocker Switch ==

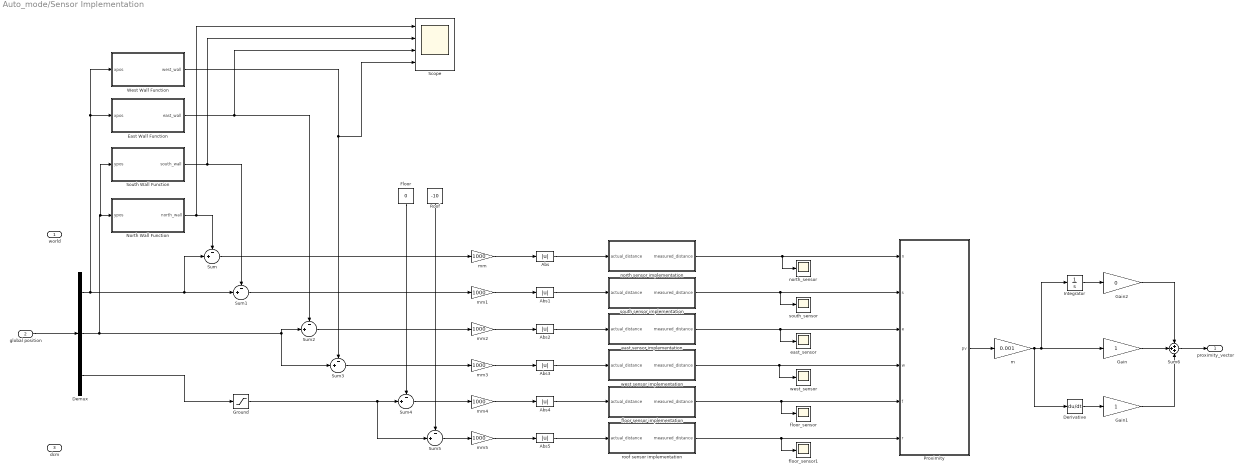
== system Auto_mode/Sensor Implementation ==
  world : Inport
  global position : Inport  Port=2
  dcm : Inport  Port=3
  Abs{,1..5} (6 alike) : Abs
  Demux : Demux  Outputs=3
  Derivative : Derivative
  East Wall Function : MATLAB Function  TreatAsAtomicUnit=on
  Floor : Constant  Value=0
  Gain : Gain
  Gain1 : Gain
  Gain2 : Gain  Gain=0
  Ground : Saturate  UpperLimit=0  LowerLimit=-100
  Integrator : Integrator
  North Wall Function : MATLAB Function  TreatAsAtomicUnit=on
  Proximity : MATLAB Function  TreatAsAtomicUnit=on
  Roof : Constant  Value=-10
  Scope : Scope  NumInputPorts=4
  South Wall Function : MATLAB Function  TreatAsAtomicUnit=on
  Sum{,1..5} (6 alike) : Sum  Inputs=-+|
  Sum6 : Sum  Inputs=+++
  West Wall Function : MATLAB Function  TreatAsAtomicUnit=on
  east sensor implementation : Subsystem
  east_sensor : Scope
  floor sensor implementation : Subsystem
  floor_sensor : Scope
  floor_sensor1 : Scope
  m : Gain  Gain=0.001
  mm{,1..5} (6 alike) : Gain  Gain=1000
  north sensor implementation : Subsystem
  north_sensor : Scope
  roof sensor implementation : Subsystem
  south sensor implementation : Subsystem
  south_sensor : Scope
  west sensor implementation : Subsystem
  west_sensor : Scope
  proximity_vector : Outport
  wires:
  global position/1 -> Demux/1
  Demux/1 -> West Wall Function/1(xpos), East Wall Function/1(xpos), Sum1/2, Sum/2
  South Wall Function/1(south_wall) -> Scope/2, Sum1/1
  Demux/2 -> South Wall Function/1(ypos), North Wall Function/1(ypos), Sum3/2, Sum2/2
  West Wall Function/1(west_wall) -> Scope/4, Sum3/1
  East Wall Function/1(east_wall) -> Scope/3, Sum2/1
  Floor/1 -> Sum4/1
  Demux/3 -> Ground/1
  Roof/1 -> Sum5/1
  Sum5/1 -> mm5/1
  Sum4/1 -> mm4/1
  Sum3/1 -> mm3/1
  Sum2/1 -> mm2/1
  Sum1/1 -> mm1/1
  Sum/1 -> mm/1
  mm/1 -> Abs/1
  mm1/1 -> Abs1/1
  mm2/1 -> Abs2/1
  mm3/1 -> Abs3/1
  mm4/1 -> Abs4/1
  mm5/1 -> Abs5/1
  Ground/1 -> Sum5/2, Sum4/2
  m/1 -> Derivative/1, Integrator/1, Gain/1
  Gain/1 -> Sum6/2
  Gain2/1 -> Sum6/1
  Proximity/1(pv) -> m/1
  Abs5/1 -> roof sensor implementation/1(actual_distance)
  Abs4/1 -> floor sensor implementation/1(actual_distance)
  Abs3/1 -> west sensor implementation/1(actual_distance)
  east sensor implementation/1(measured_distance) -> east_sensor/1, Proximity/3(e)
  north sensor implementation/1(measured_distance) -> Proximity/1(n), north_sensor/1
  Integrator/1 -> Gain2/1
  floor sensor implementation/1(measured_distance) -> floor_sensor/1, Proximity/5(f)
  south sensor implementation/1(measured_distance) -> south_sensor/1, Proximity/2(s)
  west sensor implementation/1(measured_distance) -> west_sensor/1, Proximity/4(w)
  Sum6/1 -> proximity_vector/1
  Abs2/1 -> east sensor implementation/1(actual_distance)
  Abs/1 -> north sensor implementation/1(actual_distance)
  roof sensor implementation/1(measured_distance) -> floor_sensor1/1, Proximity/6(r)
  Abs1/1 -> south sensor implementation/1(actual_distance)
  Derivative/1 -> Gain1/1
  Gain1/1 -> Sum6/3
  North Wall Function/1(north_wall) -> Scope/1, Sum/1

== system Auto_mode/Slider ==

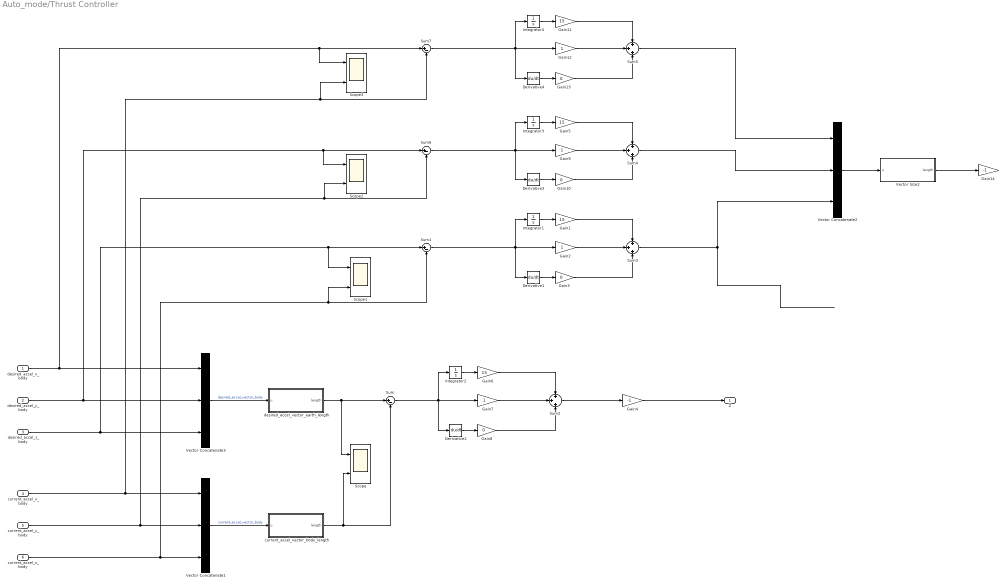
== system Auto_mode/Thrust Controller ==
  desired_accel_x_body : Inport
  desired_accel_y_body : Inport  Port=2
  desired_accel_z_body : Inport  Port=3
  current_accel_x_body : Inport  Port=4
  current_accel_y_body : Inport  Port=5
  current_accel_z_body : Inport  Port=6
  Derivative{1..4} (4 alike) : Derivative
  Gain{1,5..6,11} (4 alike) : Gain  Gain=15
  Gain{3,8,10,13} (4 alike) : Gain  Gain=0
  Gain{2,7,9,12} (4 alike) : Gain
  Gain14 : Gain  Gain=-1
  Gain4 : Gain  Gain=-1
  Integrator{1..4} (4 alike) : Integrator
  Scope{,1..3} (4 alike) : Scope  NumInputPorts=2
  Sum{,1,6..7} (4 alike) : Sum  Inputs=|+-
  Sum{2..5} (4 alike) : Sum  Inputs=+|+|+
  Vector Concatenate1 : Concatenate  NumInputs=3
  Vector Concatenate2 : Concatenate  NumInputs=3
  Vector Concatenate3 : Concatenate  NumInputs=3
  Vector Size2 : MATLAB Function  TreatAsAtomicUnit=on
  current_accel_vector_body_length : MATLAB Function  TreatAsAtomicUnit=on
  desired_accel_vector_earth_length : MATLAB Function  TreatAsAtomicUnit=on
  Z : Outport
  wires:
  Derivative2/1 -> Gain8/1
  Gain8/1 -> Sum2/3
  Gain7/1 -> Sum2/2
  Gain6/1 -> Sum2/1
  Integrator2/1 -> Gain6/1
  Vector Concatenate3/1 -> desired_accel_vector_earth_length/1(u)  "desired_accel_vector_body"
  Vector Concatenate1/1 -> current_accel_vector_body_length/1(u)  "current_accel_vector_body"
  Derivative1/1 -> Gain3/1
  Gain3/1 -> Sum3/3
  Gain2/1 -> Sum3/2
  Gain1/1 -> Sum3/1
  Integrator1/1 -> Gain1/1
  Sum1/1 -> Integrator1/1, Derivative1/1, Gain2/1
  desired_accel_z_body/1 -> Vector Concatenate3/3, Scope1/1, Sum1/1
  current_accel_z_body/1 -> Scope1/2, Sum1/2, Vector Concatenate1/3
  Derivative3/1 -> Gain10/1
  Gain10/1 -> Sum4/3
  Gain9/1 -> Sum4/2
  Gain5/1 -> Sum4/1
  Integrator3/1 -> Gain5/1
  Sum6/1 -> Integrator3/1, Derivative3/1, Gain9/1
  Sum4/1 -> Vector Concatenate2/2
  Derivative4/1 -> Gain13/1
  Gain13/1 -> Sum5/3
  Gain12/1 -> Sum5/2
  Gain11/1 -> Sum5/1
  Integrator4/1 -> Gain11/1
  Sum7/1 -> Integrator4/1, Derivative4/1, Gain12/1
  Sum5/1 -> Vector Concatenate2/1
  Vector Concatenate2/1 -> Vector Size2/1(u)
  desired_accel_y_body/1 -> Vector Concatenate3/2, Scope2/1, Sum6/1
  current_accel_y_body/1 -> Vector Concatenate1/2, Scope2/2, Sum6/2
  desired_accel_x_body/1 -> Vector Concatenate3/1, Scope3/1, Sum7/1
  current_accel_x_body/1 -> Vector Concatenate1/1, Scope3/2, Sum7/2
  Vector Size2/1(length) -> Gain14/1
  Sum3/1 -> Vector Concatenate2/3
  Sum/1 -> Derivative2/1, Integrator2/1, Gain7/1
  Sum2/1 -> Gain4/1
  desired_accel_vector_earth_length/1(length) -> Sum/1, Scope/1
  current_accel_vector_body_length/1(length) -> Sum/2, Scope/2
  Gain4/1 -> Z/1

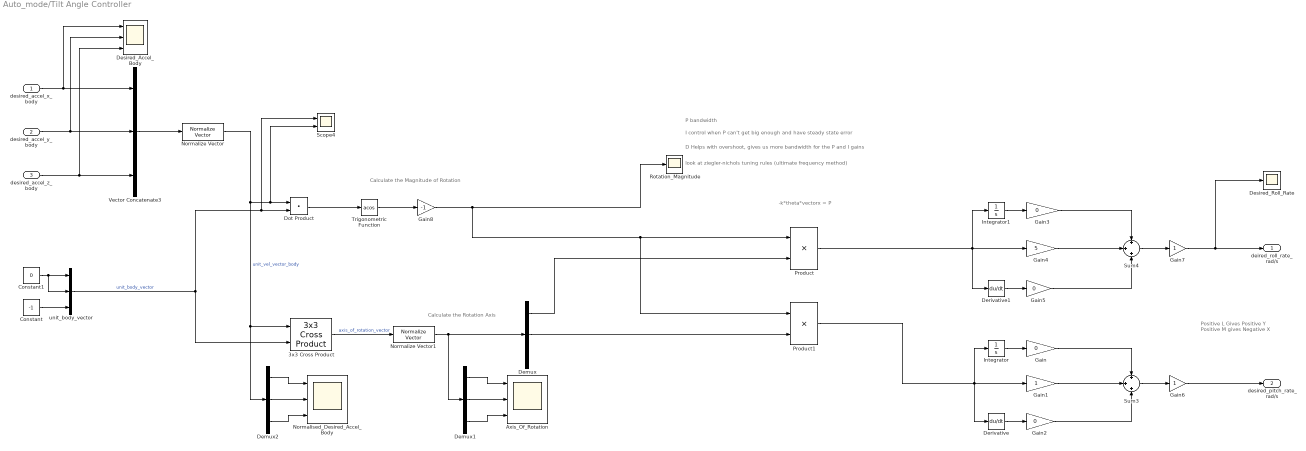
== system Auto_mode/Tilt Angle Controller ==
  note: D Helps with overshoot, gives us more bandwidth for the P and I gains
  note: I control when P can't get big enough and have steady state error
  note: P bandwidth
  note: look at ziegler-nichols tuning rules (ultimate frequency method)
  note: -k*theta*vectorx = P
  note: Calculate the Rotation Axis
  note: Calculate the Magnitude of Rotation
  note: Positive L Gives Positive Y
      | Positive M gives Negative X
  desired_accel_x_body : Inport
  desired_accel_y_body : Inport  Port=2
  desired_accel_z_body : Inport  Port=3
  3x3 Cross Product : sharedutil/3x3 Cross Product
  Axis_Of_Rotation : Scope  NumInputPorts=3
  Constant : Constant  Value=-1
  Constant1 : Constant  Value=0
  Demux : Demux  Outputs=3
  Demux1 : Demux  Outputs=3
  Demux2 : Demux  Outputs=3
  Derivative : Derivative
  Derivative1 : Derivative
  Desired_Accel_Body : Scope  NumInputPorts=3
  Desired_Roll_Rate : Scope
  Dot Product : DotProduct  InputSameDT=on  OutDataTypeStr=Inherit: Inherit via internal rule
  Gain{,2..3,5} (4 alike) : Gain  Gain=0
  Gain1 : Gain
  Gain4 : Gain  Gain=5
  Gain6 : Gain
  Gain7 : Gain
  Gain8 : Gain  Gain=-1
  Integrator : Integrator
  Integrator1 : Integrator
  "Normalised_Desired_Accel_Body " : Scope  NumInputPorts=3
  Normalize Vector : vrlib/Utilities/Normalize Vector  maxzero=0
      settings: SourceProductName=Simulink 3D Animation  SourceProductBaseCode=VR
  Normalize Vector1 : vrlib/Utilities/Normalize Vector  maxzero=0
      settings: SourceProductName=Simulink 3D Animation  SourceProductBaseCode=VR
  Product : Product
  Product1 : Product
  Rotation_Magnitude : Scope
  Scope4 : Scope  NumInputPorts=2
  Sum3 : Sum  Inputs=+|+|+
  Sum4 : Sum  Inputs=+|+|+
  Trigonometric Function : Trigonometry  Operator=acos
  Vector Concatenate3 : Concatenate  NumInputs=3
  unit_body_vector : Concatenate  NumInputs=3
  deired_roll_rate_rad/s : Outport
  desired_pitch_rate_rad/s : Outport  Port=2
  wires:
  Vector Concatenate3/1 -> Normalize Vector/1
  Normalize Vector1/1 -> Demux/1, Demux1/1
  Constant1/1 -> unit_body_vector/2, unit_body_vector/1
  Dot Product/1 -> Trigonometric Function/1
  Normalize Vector/1 -> Dot Product/1, Scope4/2, Demux2/1, 3x3 Cross Product/1  "unit_vel_vector_body"
  Constant/1 -> unit_body_vector/3
  unit_body_vector/1 -> 3x3 Cross Product/2, Dot Product/2, Scope4/1  "unit_body_vector"
  3x3 Cross Product/1 -> Normalize Vector1/1  "axis_of_rotation_vector"
  Sum3/1 -> Gain6/1
  Derivative/1 -> Gain2/1
  Gain2/1 -> Sum3/3
  Gain1/1 -> Sum3/2
  Gain/1 -> Sum3/1
  Integrator/1 -> Gain/1
  Derivative1/1 -> Gain5/1
  Gain5/1 -> Sum4/3
  Gain4/1 -> Sum4/2
  Gain3/1 -> Sum4/1
  Integrator1/1 -> Gain3/1
  Product/1 -> Integrator1/1, Derivative1/1, Gain4/1
  Product1/1 -> Derivative/1, Integrator/1, Gain1/1
  Demux/1 -> Product/2
  Demux/2 -> Product1/2
  Gain6/1 -> desired_pitch_rate_rad/s/1
  Sum4/1 -> Gain7/1
  desired_accel_y_body/1 -> Desired_Accel_Body/2, Vector Concatenate3/2
  desired_accel_x_body/1 -> Desired_Accel_Body/1, Vector Concatenate3/1
  desired_accel_z_body/1 -> Desired_Accel_Body/3, Vector Concatenate3/3
  Gain7/1 -> Desired_Roll_Rate/1, deired_roll_rate_rad/s/1
  Trigonometric Function/1 -> Gain8/1
  Demux1/2 -> Axis_Of_Rotation/2
  Demux1/1 -> Axis_Of_Rotation/1
  Demux1/3 -> Axis_Of_Rotation/3
  Demux2/2 -> "Normalised_Desired_Accel_Body "/2
  Demux2/3 -> "Normalised_Desired_Accel_Body "/3
  Demux2/1 -> "Normalised_Desired_Accel_Body "/1
  Gain8/1 -> Rotation_Magnitude/1, Product/1, Product1/1

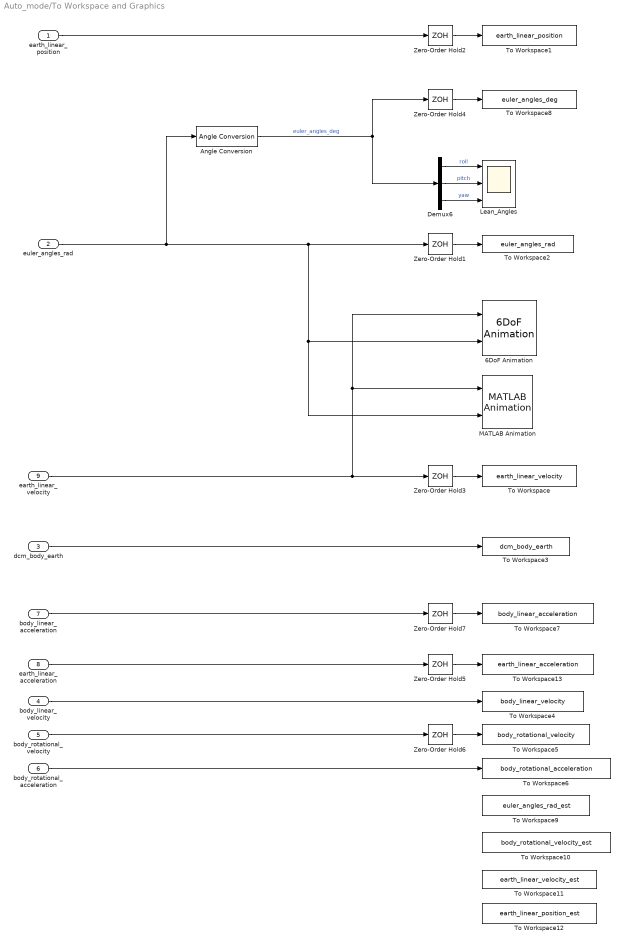
== system Auto_mode/To Workspace and Graphics ==
  earth_linear_position : Inport
  euler_angles_rad : Inport  Port=2
  dcm_body_earth : Inport  Port=3
  body_linear_velocity : Inport  Port=4
  body_rotational_velocity : Inport  Port=5
  body_rotational_acceleration : Inport  Port=6
  body_linear_acceleration : Inport  Port=7
  earth_linear_acceleration : Inport  Port=8
  earth_linear_velocity : Inport  Port=9
  6DoF Animation : aerolibanim/6DoF Animation  u1=[0 4000 -2000 2000 -5000 -3000]  u2=0.1  u3=0.1  u4=[0 0 0]  u5=Fixed position  u6=[-150 -150 -150]  u7=3  u8=off
      settings: SourceProductName=Aerospace Blockset
  Angle Conversion : aerolibconvert2/Angle Conversion  IU=rad  OU=deg
  Demux6 : Demux  Outputs=3
  Lean_Angles : Scope  NumInputPorts=3
  MATLAB Animation : aerolibanim/MATLAB Animation  Tag=Matlab Animation 6 DOF  Vehicles=1  Geometries='astredwedge.mat'  BoundingBoxCoordinates=[-50,50,-50,50,-500,500]  CameraOffset=[-150,-0,-25]  CameraViewAngle=3  SampleTime=0.2  FigurePosition=[962,42,958,981]
      settings: SourceProductName=Aerospace Blockset  SourceProductBaseCode=AE
  To Workspace : ToWorkspace  VariableName=earth_linear_velocity  SampleTime=-1
  To Workspace1 : ToWorkspace  VariableName=earth_linear_position  SampleTime=-1
  To Workspace10 : ToWorkspace  VariableName=body_rotational_velocity_est  SampleTime=-1
  To Workspace11 : ToWorkspace  VariableName=earth_linear_velocity_est  SampleTime=-1
  To Workspace12 : ToWorkspace  VariableName=earth_linear_position_est  SampleTime=-1
  To Workspace13 : ToWorkspace  VariableName=earth_linear_acceleration  SampleTime=-1
  To Workspace2 : ToWorkspace  VariableName=euler_angles_rad  SampleTime=-1
  To Workspace3 : ToWorkspace  VariableName=dcm_body_earth  SampleTime=-1
  To Workspace4 : ToWorkspace  VariableName=body_linear_velocity  SampleTime=-1
  To Workspace5 : ToWorkspace  VariableName=body_rotational_velocity  SampleTime=-1
  To Workspace6 : ToWorkspace  VariableName=body_rotational_acceleration  SampleTime=-1
  To Workspace7 : ToWorkspace  VariableName=body_linear_acceleration  SampleTime=-1
  To Workspace8 : ToWorkspace  VariableName=euler_angles_deg  SampleTime=-1
  To Workspace9 : ToWorkspace  VariableName=euler_angles_rad_est  SampleTime=-1
  Zero-Order Hold{1..7} (7 alike) : ZeroOrderHold  SampleTime=Ts
  wires:
  Angle Conversion/1 -> Zero-Order Hold4/1, Demux6/1  "euler_angles_deg"
  euler_angles_rad/1 -> 6DoF Animation/2, MATLAB Animation/2, Zero-Order Hold1/1, Angle Conversion/1
  body_rotational_velocity/1 -> Zero-Order Hold6/1
  earth_linear_position/1 -> Zero-Order Hold2/1
  Zero-Order Hold6/1 -> To Workspace5/1
  Zero-Order Hold1/1 -> To Workspace2/1
  Zero-Order Hold2/1 -> To Workspace1/1
  Zero-Order Hold4/1 -> To Workspace8/1
  body_linear_velocity/1 -> To Workspace4/1
  earth_linear_acceleration/1 -> Zero-Order Hold5/1
  dcm_body_earth/1 -> To Workspace3/1
  body_linear_acceleration/1 -> Zero-Order Hold7/1
  Zero-Order Hold5/1 -> To Workspace13/1
  Zero-Order Hold7/1 -> To Workspace7/1
  Demux6/3 -> Lean_Angles/3  "yaw"
  Demux6/2 -> Lean_Angles/2  "pitch"
  Demux6/1 -> Lean_Angles/1  "roll"
  Zero-Order Hold3/1 -> To Workspace/1
  earth_linear_velocity/1 -> 6DoF Animation/1, MATLAB Animation/1, Zero-Order Hold3/1
  body_rotational_acceleration/1 -> To Workspace6/1

== system Auto_mode/Vector Rotation Body to Earth Acceleration2 ==
  note: Convert Vector into 2nd Frame
  dcm_12 : Inport
  vector_frame1 : Inport  Port=2
  Convert Earth to body : Product  Multiplication=Matrix(*)
  vector_frame2 : Outport
  wires:
  dcm_12/1 -> Convert Earth to body/1
  vector_frame1/1 -> Convert Earth to body/2  "vector_frame1"
  Convert Earth to body/1 -> vector_frame2/1  "vector_frame2"

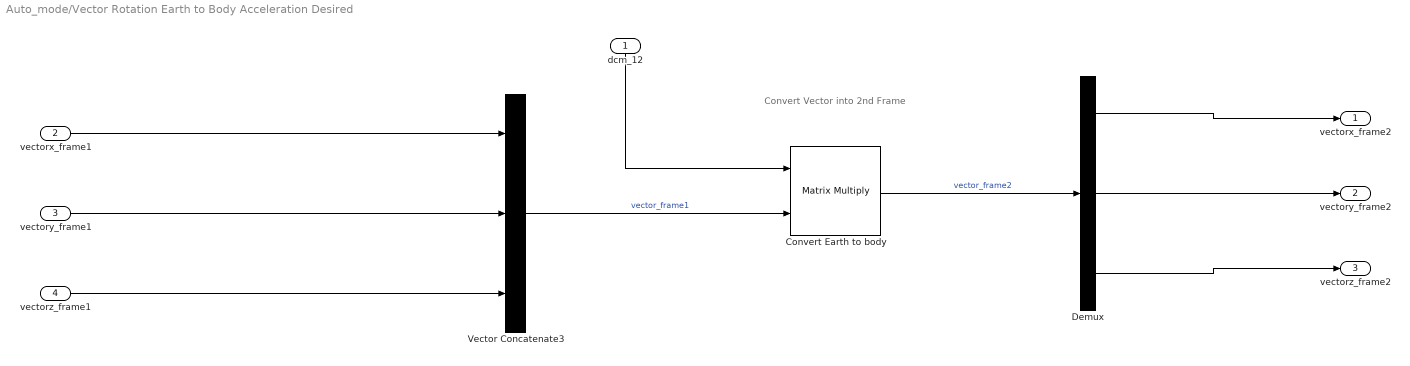
== system Auto_mode/Vector Rotation Earth to Body Acceleration Desired ==
  note: Convert Vector into 2nd Frame
  dcm_12 : Inport
  vectorx_frame1 : Inport  Port=2
  vectory_frame1 : Inport  Port=3
  vectorz_frame1 : Inport  Port=4
  Convert Earth to body : Product  Multiplication=Matrix(*)
  Demux : Demux  Outputs=3
  Vector Concatenate3 : Concatenate  NumInputs=3
  vectorx_frame2 : Outport
  vectory_frame2 : Outport  Port=2
  vectorz_frame2 : Outport  Port=3
  wires:
  vectorx_frame1/1 -> Vector Concatenate3/1
  vectory_frame1/1 -> Vector Concatenate3/2
  vectorz_frame1/1 -> Vector Concatenate3/3
  dcm_12/1 -> Convert Earth to body/1
  Vector Concatenate3/1 -> Convert Earth to body/2  "vector_frame1"
  Convert Earth to body/1 -> Demux/1  "vector_frame2"
  Demux/3 -> vectorz_frame2/1
  Demux/2 -> vectory_frame2/1
  Demux/1 -> vectorx_frame2/1

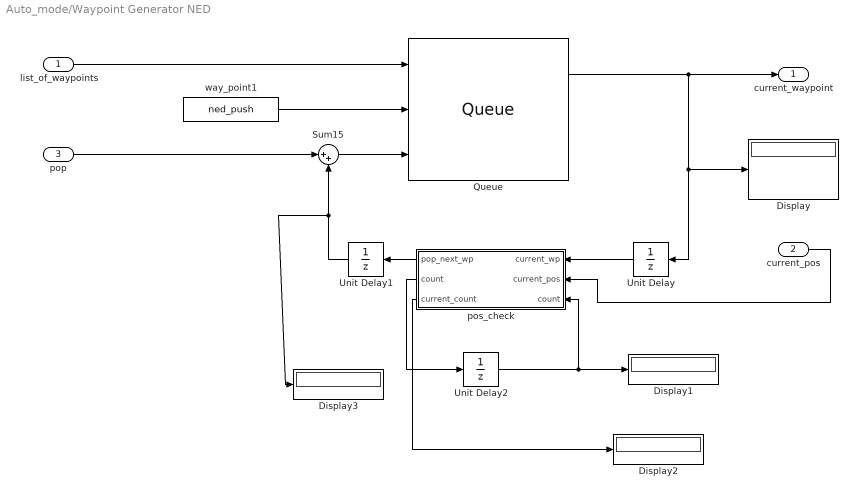
== system Auto_mode/Waypoint Generator NED ==
  list_of_waypoints : Inport
  current_pos : Inport  Port=2
  pop : Inport  Port=3
  Display{,1..3} (4 alike) : Display
  Queue : dspbuff3/Queue  depth=64  trigger=Rising edge  overflow=Ignore  pes=Ignore  eso=off  fso=off  nso=on  clr=off  clrOutport=off  adf=on
      settings: SourceProductName=DSP System Toolbox  SourceProductBaseCode=DS
  Sum15 : Sum  Inputs=|++
  Unit Delay : UnitDelay  SampleTime=-1
  Unit Delay1 : UnitDelay  SampleTime=0.1
  Unit Delay2 : UnitDelay  SampleTime=0.1
  pos_check : MATLAB Function  TreatAsAtomicUnit=on
  way_point1 : FromWorkspace  VariableName=ned_push  SampleTime=0  Interpolate=off  OutputAfterFinalValue=Holding final value
  current_waypoint : Outport
  wires:
  Unit Delay/1 -> pos_check/1(current_wp)
  Sum15/1 -> Queue/3
  Unit Delay1/1 -> Display3/1, Sum15/2
  list_of_waypoints/1 -> Queue/1
  way_point1/1 -> Queue/2
  current_pos/1 -> pos_check/2(current_pos)
  pos_check/1(pop_next_wp) -> Unit Delay1/1
  Queue/1 -> Display/1, Unit Delay/1, current_waypoint/1
  pop/1 -> Sum15/1
  pos_check/2(count) -> Unit Delay2/1
  Unit Delay2/1 -> Display1/1, pos_check/3("count ")
  pos_check/3(current_count) -> Display2/1

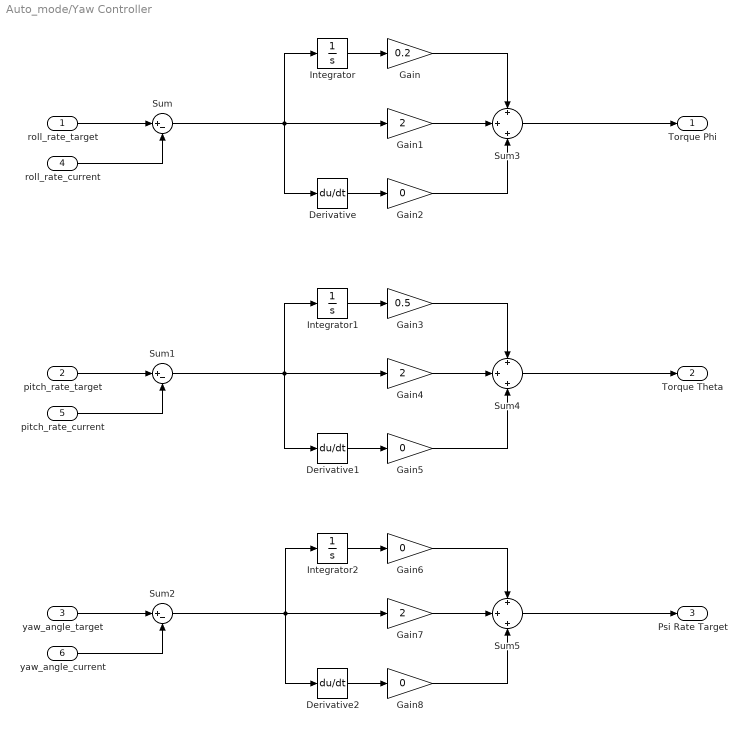
== system Auto_mode/Yaw Controller ==
  roll_rate_target : Inport
  pitch_rate_target : Inport  Port=2
  yaw_angle_target : Inport  Port=3
  roll_rate_current : Inport  Port=4
  pitch_rate_current : Inport  Port=5
  yaw_angle_current : Inport  Port=6
  Derivative : Derivative
  Derivative1 : Derivative
  Derivative2 : Derivative
  Gain : Gain  Gain=0.2
  Gain1 : Gain  Gain=2
  Gain{2,5..6,8} (4 alike) : Gain  Gain=0
  Gain3 : Gain  Gain=0.5
  Gain4 : Gain  Gain=2
  Gain7 : Gain  Gain=2
  Integrator : Integrator
  Integrator1 : Integrator
  Integrator2 : Integrator
  Sum : Sum  Inputs=|+-
  Sum1 : Sum  Inputs=|+-
  Sum2 : Sum  Inputs=|+-
  Sum3 : Sum  Inputs=+|+|+
  Sum4 : Sum  Inputs=+|+|+
  Sum5 : Sum  Inputs=+|+|+
  Torque Phi : Outport
  Torque Theta : Outport  Port=2
  Psi Rate Target : Outport  Port=3
  wires:
  roll_rate_target/1 -> Sum/1
  roll_rate_current/1 -> Sum/2
  pitch_rate_target/1 -> Sum1/1
  pitch_rate_current/1 -> Sum1/2
  yaw_angle_target/1 -> Sum2/1
  yaw_angle_current/1 -> Sum2/2
  Sum4/1 -> Torque Theta/1
  Sum3/1 -> Torque Phi/1
  Derivative/1 -> Gain2/1
  Gain2/1 -> Sum3/3
  Gain1/1 -> Sum3/2
  Gain/1 -> Sum3/1
  Integrator/1 -> Gain/1
  Sum/1 -> Derivative/1, Integrator/1, Gain1/1
  Derivative1/1 -> Gain5/1
  Gain5/1 -> Sum4/3
  Gain4/1 -> Sum4/2
  Gain3/1 -> Sum4/1
  Integrator1/1 -> Gain3/1
  Sum1/1 -> Derivative1/1, Integrator1/1, Gain4/1
  Sum5/1 -> Psi Rate Target/1
  Derivative2/1 -> Gain8/1
  Gain8/1 -> Sum5/3
  Gain7/1 -> Sum5/2
  Gain6/1 -> Sum5/1
  Integrator2/1 -> Gain6/1
  Sum2/1 -> Gain7/1, Derivative2/1, Integrator2/1

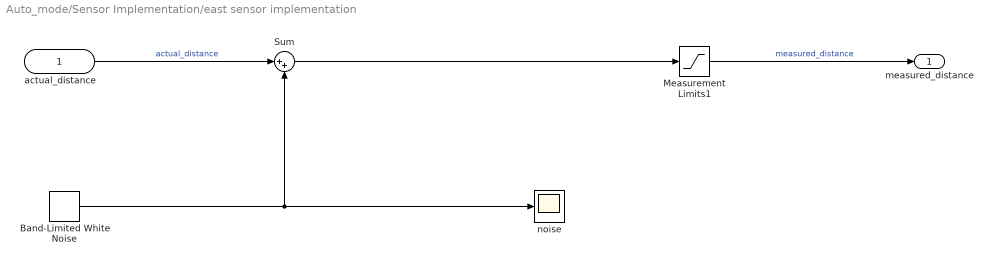
== system Auto_mode/Sensor Implementation/east sensor implementation ==
  actual_distance : Inport
  Band-Limited White Noise : simulink/Sources/Band-Limited White Noise  Cov=[0.01]  Ts=0.1  seed=[400]
  Measurement Limits1 : Saturate  UpperLimit=sensor_max_range  LowerLimit=sensor_min_range
  Sum : Sum  Inputs=|++
  noise : Scope
  measured_distance : Outport
  wires:
  actual_distance/1 -> Sum/1  "actual_distance"
  Measurement Limits1/1 -> measured_distance/1  "measured_distance"
  Band-Limited White Noise/1 -> noise/1, Sum/2
  Sum/1 -> Measurement Limits1/1

== system Auto_mode/Sensor Implementation/floor sensor implementation ==
  actual_distance : Inport
  Band-Limited White Noise : simulink/Sources/Band-Limited White Noise  Cov=[0.01]  Ts=0.1  seed=[1000]
  Measurement Limits1 : Saturate  UpperLimit=sensor_max_range  LowerLimit=sensor_min_range
  Sum : Sum  Inputs=|++
  noise : Scope
  measured_distance : Outport
  wires:
  actual_distance/1 -> Sum/1  "actual_distance"
  Measurement Limits1/1 -> measured_distance/1  "measured_distance"
  Band-Limited White Noise/1 -> noise/1, Sum/2
  Sum/1 -> Measurement Limits1/1

== system Auto_mode/Sensor Implementation/north sensor implementation ==
  actual_distance : Inport
  Band-Limited White Noise : simulink/Sources/Band-Limited White Noise  Cov=0.01  Ts=0.1  seed=[200]
  Measurement Limits : Saturate  UpperLimit=sensor_max_range  LowerLimit=sensor_min_range
  Sum : Sum  Inputs=|++
  noise : Scope
  measured_distance : Outport
  wires:
  actual_distance/1 -> Sum/1  "actual_distance"
  Measurement Limits/1 -> measured_distance/1  "measured_distance"
  Band-Limited White Noise/1 -> noise/1, Sum/2
  Sum/1 -> Measurement Limits/1

== system Auto_mode/Sensor Implementation/roof sensor implementation ==
  actual_distance : Inport
  Band-Limited White Noise : simulink/Sources/Band-Limited White Noise  Cov=[0.01]  Ts=0.1  seed=[1200]
  Measurement Limits1 : Saturate  UpperLimit=sensor_max_range  LowerLimit=sensor_min_range
  Sum : Sum  Inputs=|++
  noise : Scope
  measured_distance : Outport
  wires:
  actual_distance/1 -> Sum/1  "actual_distance"
  Measurement Limits1/1 -> measured_distance/1  "measured_distance"
  Band-Limited White Noise/1 -> noise/1, Sum/2
  Sum/1 -> Measurement Limits1/1

== system Auto_mode/Sensor Implementation/south sensor implementation ==
  actual_distance : Inport
  Band-Limited White Noise : simulink/Sources/Band-Limited White Noise  Cov=[0.01]  Ts=0.1  seed=[800]
  Measurement Limits1 : Saturate  UpperLimit=sensor_max_range  LowerLimit=sensor_min_range
  Sum : Sum  Inputs=|++
  noise : Scope
  measured_distance : Outport
  wires:
  actual_distance/1 -> Sum/1  "actual_distance"
  Measurement Limits1/1 -> measured_distance/1  "measured_distance"
  Band-Limited White Noise/1 -> noise/1, Sum/2
  Sum/1 -> Measurement Limits1/1
